simulink library "ammclib_bam_S32K3xx"  (R2016a)
(part 17 of 50)

      |   f32RampUp=round(rampsc*2^31);
      |   if f32RampUp>2^31-1
      |     f32RampUp=2^31-1;
      |     warning(['Parameter f32RampUp of ' gcb ' exceeds the fixed-point range.']);
      |   end
      |   if f32RampUp<-2^31
      |     f32RampUp=-2^31;
      |     warning(['Parameter f32RampUp of ' gcb ' exceeds the fixed-point range.']);
      |   end
      |   f32RampDown=round(rampsc*2^31);
      |   if f32RampDown>2^31-1
      |     f32RampDown=2^31-1;
      |     warning(['Parameter f32RampDown of ' gcb ' exceeds the fixed-point range.']);
      |   end
      |   if f32RampDown<-2^31
      |     f32RampDown=-2^31;
      |     warning(['Parameter f32RampDown of ' gcb ' exceeds the fixed-point range.']);
      |   end
      |   if isnan(u16NSamplesW)
      |     if ~strcmp(u16NSamplesW_bkup,'0')
      |       set_param(gcb,'u16NSamplesW','0');
      |     end
      |   else
      |     tmps=num2str(u16NSamplesW);
      |     if ~strcmp(u16NSamplesW_bkup,tmps)
      |       set_param(gcb,'u16NSamplesW',tmps);
      |     end
      |   end
      |   if isnan(u16NSamplesFW)
      |     if ~strcmp(u16NSamplesFW_bkup,'0')
      |       set_param(gcb,'u16NSamplesFW','0');
      |     end
      |   else
      |     tmps=num2str(u16NSamplesFW);
      |     if ~strcmp(u16NSamplesFW_bkup,tmps)
      |       set_param(gcb,'u16NSamplesFW',tmps);
      |     end
      |   end
      |   if isnan(f32PropGainQ)
      |     if ~strcmp(f32PropGainQ_bkup,'0')
      |       set_param(gcb,'f32PropGainQ','0');
      |     end
      |   else
      |     tmps=num2str(f32PropGainQ);
      |     if ~strcmp(f32PropGainQ_bkup,tmps)
      |       set_param(gcb,'f32PropGainQ',tmps);
      |     end
      |   end
      |   if isnan(f32IntegGainQ)
      |     if ~strcmp(f32IntegGainQ_bkup,'0')
      |       set_param(gcb,'f32IntegGainQ','0');
      |     end
      |   else
      |     tmps=num2str(f32IntegGainQ);
      |     if ~strcmp(f32IntegGainQ_bkup,tmps)
      |       set_param(gcb,'f32IntegGainQ',tmps);
      |     end
      |   end
      |   if isnan(s16PropGainShiftQ)
      |     if ~strcmp(s16PropGainShiftQ_bkup,'0')
      |       set_param(gcb,'s16PropGainShiftQ','0');
      |     end
      |   else
      |     tmps=num2str(s16PropGainShiftQ);
      |     if ~strcmp(s16PropGainShiftQ_bkup,tmps)
      |       set_param(gcb,'s16PropGainShiftQ',tmps);
      |     end
      |   end
      |   if isnan(s16IntegGainShiftQ)
      |     if ~strcmp(s16IntegGainShiftQ_bkup,'0')
      |       set_param(gcb,'s16IntegGainShiftQ','0');
      |     end
      |   else
      |     tmps=num2str(s16IntegGainShiftQ);
      |     if ~strcmp(s16IntegGainShiftQ_bkup,tmps)
      |       set_param(gcb,'s16IntegGainShiftQ',tmps);
      |     end
      |   end
      |   if isnan(f32LowerLimitQ)
      |     if ~strcmp(f32LowerLimitQ_bkup,'0')
      |       set_param(gcb,'f32LowerLimitQ','0');
      |     end
      |   else
      |     tmps=num2str(f32LowerLimitQ);
      |     if ~strcmp(f32LowerLimitQ_bkup,tmps)
      |       set_param(gcb,'f32LowerLimitQ',tmps);
      |     end
      |   end
      |   if isnan(f32UpperLimitQ)
      |     if ~strcmp(f32UpperLimitQ_bkup,'0')
      |       set_param(gcb,'f32UpperLimitQ','0');
      |     end
      |   else
      |     tmps=num2str(f32UpperLimitQ);
      |     if ~strcmp(f32UpperLimitQ_bkup,tmps)
      |       set_param(gcb,'f32UpperLimitQ',tmps);
      |     end
      |   end
      |   if isnan(f32PropGainFW)
      |     if ~strcmp(f32PropGainFW_bkup,'0')
      |       set_param(gcb,'f32PropGainFW','0');
      |     end
      |   else
      |     tmps=num2str(f32PropGainFW);
      |     if ~strcmp(f32PropGainFW_bkup,tmps)
      |       set_param(gcb,'f32PropGainFW',tmps);
      |     end
      |   end
      |   if isnan(f32IntegGainFW)
      |     if ~strcmp(f32IntegGainFW_bkup,'0')
      |       set_param(gcb,'f32IntegGainFW','0');
      |     end
      |   else
      |     tmps=num2str(f32IntegGainFW);
      |     if ~strcmp(f32IntegGainFW_bkup,tmps)
      |       set_param(gcb,'f32IntegGainFW',tmps);
      |     end
      |   end
      |   if isnan(s16PropGainShiftFW)
      |     if ~strcmp(s16PropGainShiftFW_bkup,'0')
      |       set_param(gcb,'s16PropGainShiftFW','0');
      |     end
      |   else
      |     tmps=num2str(s16PropGainShiftFW);
      |     if ~strcmp(s16PropGainShiftFW_bkup,tmps)
      |       set_param(gcb,'s16PropGainShiftFW',tmps);
      |     end
      |   end
      |   if isnan(s16IntegGainShiftFW)
      |     if ~strcmp(s16IntegGainShiftFW_bkup,'0')
      |       set_param(gcb,'s16IntegGainShiftFW','0');
      |     end
      |   else
      |     tmps=num2str(s16IntegGainShiftFW);
      |     if ~strcmp(s16IntegGainShiftFW_bkup,tmps)
      |       set_param(gcb,'s16IntegGainShiftFW',tmps);
      |     end
      |   end
      |   if isnan(f32LowerLimitFW)
      |     if ~strcmp(f32LowerLimitFW_bkup,'0')
      |       set_param(gcb,'f32LowerLimitFW','0');
      |     end
      |   else
      |     tmps=num2str(f32LowerLimitFW);
      |     if ~strcmp(f32LowerLimitFW_bkup,tmps)
      |       set_param(gcb,'f32LowerLimitFW',tmps);
      |     end
      |   end
      |   if isnan(f32UpperLimitFW)
      |     if ~strcmp(f32UpperLimitFW_bkup,'0')
      |       set_param(gcb,'f32UpperLimitFW','0');
      |     end
      |   else
      |     tmps=num2str(f32UpperLimitFW);
      |     if ~strcmp(f32UpperLimitFW_bkup,tmps)
      |       set_param(gcb,'f32UpperLimitFW',tmps);
      |     end
      |   end
      |   if isnan(f32RampUp)
      |     if ~strcmp(f32RampUp_bkup,'0')
      |       set_param(gcb,'f32RampUp','0');
      |     end
      |   else
      |     tmps=num2str(f32RampUp);
      |     if ~strcmp(f32RampUp_bkup,tmps)
      |       set_param(gcb,'f32RampUp',tmps);
      |     end
      |   end
      |   if isnan(f32RampDown)
      |     if ~strcmp(f32RampDown_bkup,'0')
      |       set_param(gcb,'f32RampDown','0');
      |     end
      |   else
      |     tmps=num2str(f32RampDown);
      |     if ~strcmp(f32RampDown_bkup,tmps)
      |       set_param(gcb,'f32RampDown',tmps);
      |     end
      |   end
      | end
      mask Callback autoCalcEn:
      | maskStr=get_param(gcb,'showStates');
      | if strcmp(maskStr,'Hide (faster execution)')
      |   p=Simulink.Mask.get(gcb);
      |   autoCalcEn=get_param(gcb,'autoCalcEn');
      |   hintText=p.getDialogControl('timeHint');
      |   if strcmp(autoCalcEn,'on')
      |     param=p.getParameter('iscale');
      |     if strcmp(param.Enabled,'off')
      |       SampleTime=Simulink.data.evalinGlobal(bdroot,get_param(gcb,'SampleTime'));
      |       if SampleTime==-1
      |         SampleTime=str2double(get_param(gcb,'SampleTime_1'));
      |         if isnan(SampleTime)
      |           hintText.Prompt=['Note: Implementation parameters cannot be calculated yet because the block''s inherited sample time is unknown. Simulink will update the sample time when you run the simulation.'];
      |         else
      |           hintText.Prompt=['Caution: Implementation parameters depend on inherited sample time. Make sure that the sample time of the block''s inputs corresponds to the sampling period in the target application.'];
      |         end
      |       else
      |         hintText.Prompt='Caution: Implementation parameters depend on the sample time. Make sure that the simulation time step corresponds to the sampling period in the target application.';
      |       end
      |       p=Simulink.Mask.get(gcb);
      |       param=p.getParameter('wf0');
      |       param.set('Enabled','on');
      |       param=p.getParameter('wksi');
      |       param.set('Enabled','on');
      |       param=p.getParameter('J');
      |       param.set('Enabled','on');
      |       param=p.getParameter('Kt');
      |       param.set('Enabled','on');
      |       param=p.getParameter('lambdaW');
      |       param.set('Enabled','on');
      |       param=p.getParameter('lambdaFW');
      |       param.set('Enabled','on');
      |       param=p.getParameter('Idmax');
      |       param.set('Enabled','on');
      |       param=p.getParameter('ramprpm');
      |       param.set('Enabled','on');
      |       param=p.getParameter('mechspeed');
      |       param.set('Enabled','on');
      |       param=p.getParameter('polepairs');
      |       param.set('Enabled','on');
      |       param=p.getParameter('uscale');
      |       param.set('Enabled','on');
      |       param=p.getParameter('iscale');
      |       param.set('Enabled','on');
      |     else
      |       SampleTime=Simulink.data.evalinGlobal(bdroot,get_param(gcb,'SampleTime'));
      |       if SampleTime==-1
      |         SampleTime=str2double(get_param(gcb,'SampleTime_1'));
      |       end
      |     end
      |     u16NSamplesW_bkup=get_param(gcb,'u16NSamplesW');
      |     u16NSamplesFW_bkup=get_param(gcb,'u16NSamplesFW');
      |     f32PropGainQ_bkup=get_param(gcb,'f32PropGainQ');
      |     f32IntegGainQ_bkup=get_param(gcb,'f32IntegGainQ');
      |     s16PropGainShiftQ_bkup=get_param(gcb,'s16PropGainShiftQ');
      |     s16IntegGainShiftQ_bkup=get_param(gcb,'s16IntegGainShiftQ');
      |     f32LowerLimitQ_bkup=get_param(gcb,'f32LowerLimitQ');
      |     f32UpperLimitQ_bkup=get_param(gcb,'f32UpperLimitQ');
      |     f32PropGainFW_bkup=get_param(gcb,'f32PropGainFW');
      |     f32IntegGainFW_bkup=get_param(gcb,'f32IntegGainFW');
      |     s16PropGainShiftFW_bkup=get_param(gcb,'s16PropGainShiftFW');
      |     s16IntegGainShiftFW_bkup=get_param(gcb,'s16IntegGainShiftFW');
      |     f32LowerLimitFW_bkup=get_param(gcb,'f32LowerLimitFW');
      |     f32UpperLimitFW_bkup=get_param(gcb,'f32UpperLimitFW');
      |     f32RampUp_bkup=get_param(gcb,'f32RampUp');
      |     f32RampDown_bkup=get_param(gcb,'f32RampDown');
      |     wf0=Simulink.data.evalinGlobal(bdroot,get_param(gcb,'wf0'));
      |     wksi=Simulink.data.evalinGlobal(bdroot,get_param(gcb,'wksi'));
      |     J=Simulink.data.evalinGlobal(bdroot,get_param(gcb,'J'));
      |     Kt=Simulink.data.evalinGlobal(bdroot,get_param(gcb,'Kt'));
      |     lambdaW=Simulink.data.evalinGlobal(bdroot,get_param(gcb,'lambdaW'));
      |     lambdaFW=Simulink.data.evalinGlobal(bdroot,get_param(gcb,'lambdaFW'));
      |     Idmax=Simulink.data.evalinGlobal(bdroot,get_param(gcb,'Idmax'));
      |     ramprpm=Simulink.data.evalinGlobal(bdroot,get_param(gcb,'ramprpm'));
      |     mechspeed=Simulink.data.evalinGlobal(bdroot,get_param(gcb,'mechspeed'));
      |     polepairs=Simulink.data.evalinGlobal(bdroot,get_param(gcb,'polepairs'));
      |     uscale=Simulink.data.evalinGlobal(bdroot,get_param(gcb,'uscale'));
      |     iscale=Simulink.data.evalinGlobal(bdroot,get_param(gcb,'iscale'));
      |     if (wf0<=0)
      |       warning('Natural frequency f0 must be positive.');
      |     end
      |     if (wksi<=0)
      |       warning('Current loop attenuation must be positive.');
      |     end
      |     if (wksi>1)
      |       warning('Current loop attenuation must not exceed 1.');
      |     end
      |     if (J<=0)
      |       warning('Moment of inertia J must be positive.');
      |     end
      |     if (Kt<=0)
      |       warning('Torque constant Kt must be positive.');
      |     end
      |     if (lambdaW<0)
      |       warning('MA filter smoothing factor must be in the range 0..1.');
      |     end
      |     if (lambdaW>1)
      |       warning('MA filter smoothing factor must be in the range 0..1.');
      |     end
      |     if (lambdaFW<0)
      |       warning('MA filter smoothing factor must be in the range 0..1.');
      |     end
      |     if (lambdaFW>1)
      |       warning('MA filter smoothing factor must be in the range 0..1.');
      |     end
      |     if (mechspeed<=0)
      |       warning('Max. speed must be positive.');
      |     end
      |     if (polepairs<1)
      |       warning('Number of pole pairs must be a natural number (1, 2, 3, ...).');
      |     end
      |     if (round(polepairs)~=polepairs)
      |       warning('Number of pole pairs must be a natural number (1, 2, 3, ...).');
      |     end
      |     if (uscale<=0)
      |       warning('U_max must be positive.');
      |     end
      |     if (iscale<=0)
      |       warning('I_max must be positive.');
      |     end
      |     w0=6.283185307179586*wf0;
      |     pgain=2.0*wksi*w0*J/Kt;
      |     igain=w0*w0*J/Kt;
      |     wmax=polepairs*mechspeed*0.1047197551196598;
      |     kpf=pgain*wmax/iscale;
      |     s16PropGainShiftQ=ceil(log2(abs(kpf)));
      |     if s16PropGainShiftQ<-31
      |       s16PropGainShiftQ=-31;
      |     end
      |     if s16PropGainShiftQ>31
      |       s16PropGainShiftQ=31;
      |       warning(['Parameter s16PropGainShiftQ of ' gcb ' exceeds the fixed-point range.']);
      |     end
      |     f32PropGainQ=round(kpf*2^(-s16PropGainShiftQ)*2^31);
      |     if f32PropGainQ>2^31-1
      |       f32PropGainQ=2^31-1;
      |       warning(['Parameter f32PropGainQ of ' gcb ' exceeds the fixed-point range.']);
      |     end
      |     if f32PropGainQ<-2^31
      |       f32PropGainQ=-2^31;
      |       warning(['Parameter f32PropGainQ of ' gcb ' exceeds the fixed-point range.']);
      |     end
      |     kif=igain*SampleTime*0.5*wmax/iscale;
      |     s16IntegGainShiftQ=ceil(log2(abs(kif)));
      |     if s16IntegGainShiftQ<-31
      |       s16IntegGainShiftQ=-31;
      |     end
      |     if s16IntegGainShiftQ>31
      |       s16IntegGainShiftQ=31;
      |       warning(['Parameter s16IntegGainShiftQ of ' gcb ' exceeds the fixed-point range.']);
      |     end
      |     f32IntegGainQ=round(kif*2^(-s16IntegGainShiftQ)*2^31);
      |     if f32IntegGainQ>2^31-1
      |       f32IntegGainQ=2^31-1;
      |       warning(['Parameter f32IntegGainQ of ' gcb ' exceeds the fixed-point range.']);
      |     end
      |     if f32IntegGainQ<-2^31
      |       f32IntegGainQ=-2^31;
      |       warning(['Parameter f32IntegGainQ of ' gcb ' exceeds the fixed-point range.']);
      |     end
      |     f32LowerLimitQ=-2147483648;
      |     f32UpperLimitQ=2147483647;
      |     fwkpf=0.9*pgain*wmax/iscale;
      |     s16PropGainShiftFW=ceil(log2(abs(fwkpf)));
      |     if s16PropGainShiftFW<-31
      |       s16PropGainShiftFW=-31;
      |     end
      |     if s16PropGainShiftFW>31
      |       s16PropGainShiftFW=31;
      |       warning(['Parameter s16PropGainShiftFW of ' gcb ' exceeds the fixed-point range.']);
      |     end
      |     f32PropGainFW=round(fwkpf*2^(-s16PropGainShiftFW)*2^31);
      |     if f32PropGainFW>2^31-1
      |       f32PropGainFW=2^31-1;
      |       warning(['Parameter f32PropGainFW of ' gcb ' exceeds the fixed-point range.']);
      |     end
      |     if f32PropGainFW<-2^31
      |       f32PropGainFW=-2^31;
      |       warning(['Parameter f32PropGainFW of ' gcb ' exceeds the fixed-point range.']);
      |     end
      |     s16IntegGainShiftFW=s16IntegGainShiftQ;
      |     f32IntegGainFW=f32IntegGainQ;
      |     if (Idmax<0)
      |       iratio=abs(Idmax)/iscale;
      |       if (abs(iratio) > 1)
      |         iratio = 0;
      |       end
      |       lowlim=0.3183098861837907*acos(iratio)-0.5;
      |     else
      |       lowlim=0.0;
      |     end
      |     f32LowerLimitFW=round(lowlim*2^31);
      |     if f32LowerLimitFW>2^31-1
      |       f32LowerLimitFW=2^31-1;
      |       warning(['Parameter f32LowerLimitFW of ' gcb ' exceeds the fixed-point range.']);
      |     end
      |     if f32LowerLimitFW<-2^31
      |       f32LowerLimitFW=-2^31;
      |       warning(['Parameter f32LowerLimitFW of ' gcb ' exceeds the fixed-point range.']);
      |     end
      |     f32UpperLimitFW=0;
      |     u16NSamplesW=round(log2(1.0/abs(lambdaW)));
      |     if u16NSamplesW>31
      |       u16NSamplesW=31;
      |     end
      |     if u16NSamplesW<0
      |       u16NSamplesW=0;
      |     end
      |     u16NSamplesFW=round(log2(1.0/abs(lambdaFW)));
      |     if u16NSamplesFW>31
      |       u16NSamplesFW=31;
      |     end
      |     if u16NSamplesFW<0
      |       u16NSamplesFW=0;
      |     end
      |     rampsc=polepairs*abs(ramprpm)*0.1047197551196598/wmax;
      |     f32RampUp=round(rampsc*2^31);
      |     if f32RampUp>2^31-1
      |       f32RampUp=2^31-1;
      |       warning(['Parameter f32RampUp of ' gcb ' exceeds the fixed-point range.']);
      |     end
      |     if f32RampUp<-2^31
      |       f32RampUp=-2^31;
      |       warning(['Parameter f32RampUp of ' gcb ' exceeds the fixed-point range.']);
      |     end
      |     f32RampDown=round(rampsc*2^31);
      |     if f32RampDown>2^31-1
      |       f32RampDown=2^31-1;
      |       warning(['Parameter f32RampDown of ' gcb ' exceeds the fixed-point range.']);
      |     end
      |     if f32RampDown<-2^31
      |       f32RampDown=-2^31;
      |       warning(['Parameter f32RampDown of ' gcb ' exceeds the fixed-point range.']);
      |     end
      |     if isnan(u16NSamplesW)
      |       if ~strcmp(u16NSamplesW_bkup,'0')
      |         set_param(gcb,'u16NSamplesW','0');
      |       end
      |     else
      |       tmps=num2str(u16NSamplesW);
      |       if ~strcmp(u16NSamplesW_bkup,tmps)
      |         set_param(gcb,'u16NSamplesW',tmps);
      |       end
      |     end
      |     if isnan(u16NSamplesFW)
      |       if ~strcmp(u16NSamplesFW_bkup,'0')
      |         set_param(gcb,'u16NSamplesFW','0');
      |       end
      |     else
      |       tmps=num2str(u16NSamplesFW);
      |       if ~strcmp(u16NSamplesFW_bkup,tmps)
      |         set_param(gcb,'u16NSamplesFW',tmps);
      |       end
      |     end
      |     if isnan(f32PropGainQ)
      |       if ~strcmp(f32PropGainQ_bkup,'0')
      |         set_param(gcb,'f32PropGainQ','0');
      |       end
      |     else
      |       tmps=num2str(f32PropGainQ);
      |       if ~strcmp(f32PropGainQ_bkup,tmps)
      |         set_param(gcb,'f32PropGainQ',tmps);
      |       end
      |     end
      |     if isnan(f32IntegGainQ)
      |       if ~strcmp(f32IntegGainQ_bkup,'0')
      |         set_param(gcb,'f32IntegGainQ','0');
      |       end
      |     else
      |       tmps=num2str(f32IntegGainQ);
      |       if ~strcmp(f32IntegGainQ_bkup,tmps)
      |         set_param(gcb,'f32IntegGainQ',tmps);
      |       end
      |     end
      |     if isnan(s16PropGainShiftQ)
      |       if ~strcmp(s16PropGainShiftQ_bkup,'0')
      |         set_param(gcb,'s16PropGainShiftQ','0');
      |       end
      |     else
      |       tmps=num2str(s16PropGainShiftQ);
      |       if ~strcmp(s16PropGainShiftQ_bkup,tmps)
      |         set_param(gcb,'s16PropGainShiftQ',tmps);
      |       end
      |     end
      |     if isnan(s16IntegGainShiftQ)
      |       if ~strcmp(s16IntegGainShiftQ_bkup,'0')
      |         set_param(gcb,'s16IntegGainShiftQ','0');
      |       end
      |     else
      |       tmps=num2str(s16IntegGainShiftQ);
      |       if ~strcmp(s16IntegGainShiftQ_bkup,tmps)
      |         set_param(gcb,'s16IntegGainShiftQ',tmps);
      |       end
      |     end
      |     if isnan(f32LowerLimitQ)
      |       if ~strcmp(f32LowerLimitQ_bkup,'0')
      |         set_param(gcb,'f32LowerLimitQ','0');
      |       end
      |     else
      |       tmps=num2str(f32LowerLimitQ);
      |       if ~strcmp(f32LowerLimitQ_bkup,tmps)
      |         set_param(gcb,'f32LowerLimitQ',tmps);
      |       end
      |     end
      |     if isnan(f32UpperLimitQ)
      |       if ~strcmp(f32UpperLimitQ_bkup,'0')
      |         set_param(gcb,'f32UpperLimitQ','0');
      |       end
      |     else
      |       tmps=num2str(f32UpperLimitQ);
      |       if ~strcmp(f32UpperLimitQ_bkup,tmps)
      |         set_param(gcb,'f32UpperLimitQ',tmps);
      |       end
      |     end
      |     if isnan(f32PropGainFW)
      |       if ~strcmp(f32PropGainFW_bkup,'0')
      |         set_param(gcb,'f32PropGainFW','0');
      |       end
      |     else
      |       tmps=num2str(f32PropGainFW);
      |       if ~strcmp(f32PropGainFW_bkup,tmps)
      |         set_param(gcb,'f32PropGainFW',tmps);
      |       end
      |     end
      |     if isnan(f32IntegGainFW)
      |       if ~strcmp(f32IntegGainFW_bkup,'0')
      |         set_param(gcb,'f32IntegGainFW','0');
      |       end
      |     else
      |       tmps=num2str(f32IntegGainFW);
      |       if ~strcmp(f32IntegGainFW_bkup,tmps)
      |         set_param(gcb,'f32IntegGainFW',tmps);
      |       end
      |     end
      |     if isnan(s16PropGainShiftFW)
      |       if ~strcmp(s16PropGainShiftFW_bkup,'0')
      |         set_param(gcb,'s16PropGainShiftFW','0');
      |       end
      |     else
      |       tmps=num2str(s16PropGainShiftFW);
      |       if ~strcmp(s16PropGainShiftFW_bkup,tmps)
      |         set_param(gcb,'s16PropGainShiftFW',tmps);
      |       end
      |     end
      |     if isnan(s16IntegGainShiftFW)
      |       if ~strcmp(s16IntegGainShiftFW_bkup,'0')
      |         set_param(gcb,'s16IntegGainShiftFW','0');
      |       end
      |     else
      |       tmps=num2str(s16IntegGainShiftFW);
      |       if ~strcmp(s16IntegGainShiftFW_bkup,tmps)
      |         set_param(gcb,'s16IntegGainShiftFW',tmps);
      |       end
      |     end
      |     if isnan(f32LowerLimitFW)
      |       if ~strcmp(f32LowerLimitFW_bkup,'0')
      |         set_param(gcb,'f32LowerLimitFW','0');
      |       end
      |     else
      |       tmps=num2str(f32LowerLimitFW);
      |       if ~strcmp(f32LowerLimitFW_bkup,tmps)
      |         set_param(gcb,'f32LowerLimitFW',tmps);
      |       end
      |     end
      |     if isnan(f32UpperLimitFW)
      |       if ~strcmp(f32UpperLimitFW_bkup,'0')
      |         set_param(gcb,'f32UpperLimitFW','0');
      |       end
      |     else
      |       tmps=num2str(f32UpperLimitFW);
      |       if ~strcmp(f32UpperLimitFW_bkup,tmps)
      |         set_param(gcb,'f32UpperLimitFW',tmps);
      |       end
      |     end
      |     if isnan(f32RampUp)
      |       if ~strcmp(f32RampUp_bkup,'0')
      |         set_param(gcb,'f32RampUp','0');
      |       end
      |     else
      |       tmps=num2str(f32RampUp);
      |       if ~strcmp(f32RampUp_bkup,tmps)
      |         set_param(gcb,'f32RampUp',tmps);
      |       end
      |     end
      |     if isnan(f32RampDown)
      |       if ~strcmp(f32RampDown_bkup,'0')
      |         set_param(gcb,'f32RampDown','0');
      |       end
      |     else
      |       tmps=num2str(f32RampDown);
      |       if ~strcmp(f32RampDown_bkup,tmps)
      |         set_param(gcb,'f32RampDown',tmps);
      |       end
      |     end
      |   else
      |     param=p.getParameter('iscale');
      |     if strcmp(param.Enabled,'on')
      |       hintText.Prompt='Caution: Implementation parameters are fixed.';
      |       p=Simulink.Mask.get(gcb);
      |       param=p.getParameter('wf0');
      |       param.set('Enabled','off');
      |       param=p.getParameter('wksi');
      |       param.set('Enabled','off');
      |       param=p.getParameter('J');
      |       param.set('Enabled','off');
      |       param=p.getParameter('Kt');
      |       param.set('Enabled','off');
      |       param=p.getParameter('lambdaW');
      |       param.set('Enabled','off');
      |       param=p.getParameter('lambdaFW');
      |       param.set('Enabled','off');
      |       param=p.getParameter('Idmax');
      |       param.set('Enabled','off');
      |       param=p.getParameter('ramprpm');
      |       param.set('Enabled','off');
      |       param=p.getParameter('mechspeed');
      |       param.set('Enabled','off');
      |       param=p.getParameter('polepairs');
      |       param.set('Enabled','off');
      |       param=p.getParameter('uscale');
      |       param.set('Enabled','off');
      |       param=p.getParameter('iscale');
      |       param.set('Enabled','off');
      |     end
      |   end
      | end
      mask DialogControl CompBut Prompt: Recalculate sample times
      mask DialogControl CompBut Tooltip: Simulink updates the sample times of all blocks when the simulation is run. This button will update the sample times now.
      mask DialogControl CompBut Callback:
      | btn=questdlg('This will apply all changes in all open dialog boxes and update the schematic. Do you want to proceed?','Apply all changes','Continue','Cancel','Continue');
      | if strcmp(btn,'Continue')
      |   dlgs=DAStudio.ToolRoot.getOpenDialogs;
      |   for i=1:length(dlgs)
      |     dlgs(i).apply;
      |   end
      |   try
      |     SampleTime_1=str2double(get_param(gcb,'SampleTime_1'));
      |     ts=Simulink.Block.getSampleTimes(gcb);
      |     ts=ts(1).Value(1);
      |     if (SampleTime_1 ~= ts)
      |       SampleTime_1=ts;
      |       set_param(gcb,'SampleTime_1',num2str(ts));
      |       autoCalcEn=get_param(gcb,'autoCalcEn');
      |       if strcmp(autoCalcEn,'on')
      |         SampleTime=Simulink.data.evalinGlobal(bdroot,get_param(gcb,'SampleTime'));
      |         p=Simulink.Mask.get(gcb);
      |         hintText=p.getDialogControl('timeHint');
      |         if SampleTime==-1
      |           SampleTime=SampleTime_1;
      |           hintText.Prompt='Caution: Implementation parameters depend on inherited sample time. Make sure that the sample time of the block''s inputs corresponds to the sampling period in the target application.';
      |         else
      |           hintText.Prompt='Caution: Implementation parameters depend on the sample time. Make sure that the simulation time step corresponds to the sampling period in the target application.';
      |         end
      |         u16NSamplesW_bkup=get_param(gcb,'u16NSamplesW');
      |         u16NSamplesFW_bkup=get_param(gcb,'u16NSamplesFW');
      |         f32PropGainQ_bkup=get_param(gcb,'f32PropGainQ');
      |         f32IntegGainQ_bkup=get_param(gcb,'f32IntegGainQ');
      |         s16PropGainShiftQ_bkup=get_param(gcb,'s16PropGainShiftQ');
      |         s16IntegGainShiftQ_bkup=get_param(gcb,'s16IntegGainShiftQ');
      |         f32LowerLimitQ_bkup=get_param(gcb,'f32LowerLimitQ');
      |         f32UpperLimitQ_bkup=get_param(gcb,'f32UpperLimitQ');
      |         f32PropGainFW_bkup=get_param(gcb,'f32PropGainFW');
      |         f32IntegGainFW_bkup=get_param(gcb,'f32IntegGainFW');
      |         s16PropGainShiftFW_bkup=get_param(gcb,'s16PropGainShiftFW');
      |         s16IntegGainShiftFW_bkup=get_param(gcb,'s16IntegGainShiftFW');
      |         f32LowerLimitFW_bkup=get_param(gcb,'f32LowerLimitFW');
      |         f32UpperLimitFW_bkup=get_param(gcb,'f32UpperLimitFW');
      |         f32RampUp_bkup=get_param(gcb,'f32RampUp');
      |         f32RampDown_bkup=get_param(gcb,'f32RampDown');
      |         wf0=Simulink.data.evalinGlobal(bdroot,get_param(gcb,'wf0'));
      |         wksi=Simulink.data.evalinGlobal(bdroot,get_param(gcb,'wksi'));
      |         J=Simulink.data.evalinGlobal(bdroot,get_param(gcb,'J'));
      |         Kt=Simulink.data.evalinGlobal(bdroot,get_param(gcb,'Kt'));
      |         lambdaW=Simulink.data.evalinGlobal(bdroot,get_param(gcb,'lambdaW'));
      |         lambdaFW=Simulink.data.evalinGlobal(bdroot,get_param(gcb,'lambdaFW'));
      |         Idmax=Simulink.data.evalinGlobal(bdroot,get_param(gcb,'Idmax'));
      |         ramprpm=Simulink.data.evalinGlobal(bdroot,get_param(gcb,'ramprpm'));
      |         mechspeed=Simulink.data.evalinGlobal(bdroot,get_param(gcb,'mechspeed'));
      |         polepairs=Simulink.data.evalinGlobal(bdroot,get_param(gcb,'polepairs'));
      |         uscale=Simulink.data.evalinGlobal(bdroot,get_param(gcb,'uscale'));
      |         iscale=Simulink.data.evalinGlobal(bdroot,get_param(gcb,'iscale'));
      |         if (wf0<=0)
      |           warning('Natural frequency f0 must be positive.');
      |         end
      |         if (wksi<=0)
      |           warning('Current loop attenuation must be positive.');
      |         end
      |         if (wksi>1)
      |           warning('Current loop attenuation must not exceed 1.');
      |         end
      |         if (J<=0)
      |           warning('Moment of inertia J must be positive.');
      |         end
      |         if (Kt<=0)
      |           warning('Torque constant Kt must be positive.');
      |         end
      |         if (lambdaW<0)
      |           warning('MA filter smoothing factor must be in the range 0..1.');
      |         end
      |         if (lambdaW>1)
      |           warning('MA filter smoothing factor must be in the range 0..1.');
      |         end
      |         if (lambdaFW<0)
      |           warning('MA filter smoothing factor must be in the range 0..1.');
      |         end
      |         if (lambdaFW>1)
      |           warning('MA filter smoothing factor must be in the range 0..1.');
      |         end
      |         if (mechspeed<=0)
      |           warning('Max. speed must be positive.');
      |         end
      |         if (polepairs<1)
      |           warning('Number of pole pairs must be a natural number (1, 2, 3, ...).');
      |         end
      |         if (round(polepairs)~=polepairs)
      |           warning('Number of pole pairs must be a natural number (1, 2, 3, ...).');
      |         end
      |         if (uscale<=0)
      |           warning('U_max must be positive.');
      |         end
      |         if (iscale<=0)
      |           warning('I_max must be positive.');
      |         end
      |         w0=6.283185307179586*wf0;
      |         pgain=2.0*wksi*w0*J/Kt;
      |         igain=w0*w0*J/Kt;
      |         wmax=polepairs*mechspeed*0.1047197551196598;
      |         kpf=pgain*wmax/iscale;
      |         s16PropGainShiftQ=ceil(log2(abs(kpf)));
      |         if s16PropGainShiftQ<-31
      |           s16PropGainShiftQ=-31;
      |         end
      |         if s16PropGainShiftQ>31
      |           s16PropGainShiftQ=31;
      |           warning(['Parameter s16PropGainShiftQ of ' gcb ' exceeds the fixed-point range.']);
      |         end
      |         f32PropGainQ=round(kpf*2^(-s16PropGainShiftQ)*2^31);
      |         if f32PropGainQ>2^31-1
      |           f32PropGainQ=2^31-1;
      |           warning(['Parameter f32PropGainQ of ' gcb ' exceeds the fixed-point range.']);
      |         end
      |         if f32PropGainQ<-2^31
      |           f32PropGainQ=-2^31;
      |           warning(['Parameter f32PropGainQ of ' gcb ' exceeds the fixed-point range.']);
      |         end
      |         kif=igain*SampleTime*0.5*wmax/iscale;
      |         s16IntegGainShiftQ=ceil(log2(abs(kif)));
      |         if s16IntegGainShiftQ<-31
      |           s16IntegGainShiftQ=-31;
      |         end
      |         if s16IntegGainShiftQ>31
      |           s16IntegGainShiftQ=31;
      |           warning(['Parameter s16IntegGainShiftQ of ' gcb ' exceeds the fixed-point range.']);
      |         end
      |         f32IntegGainQ=round(kif*2^(-s16IntegGainShiftQ)*2^31);
      |         if f32IntegGainQ>2^31-1
      |           f32IntegGainQ=2^31-1;
      |           warning(['Parameter f32IntegGainQ of ' gcb ' exceeds the fixed-point range.']);
      |         end
      |         if f32IntegGainQ<-2^31
      |           f32IntegGainQ=-2^31;
      |           warning(['Parameter f32IntegGainQ of ' gcb ' exceeds the fixed-point range.']);
      |         end
      |         f32LowerLimitQ=-2147483648;
      |         f32UpperLimitQ=2147483647;
      |         fwkpf=0.9*pgain*wmax/iscale;
      |         s16PropGainShiftFW=ceil(log2(abs(fwkpf)));
      |         if s16PropGainShiftFW<-31
      |           s16PropGainShiftFW=-31;
      |         end
      |         if s16PropGainShiftFW>31
      |           s16PropGainShiftFW=31;
      |           warning(['Parameter s16PropGainShiftFW of ' gcb ' exceeds the fixed-point range.']);
      |         end
      |         f32PropGainFW=round(fwkpf*2^(-s16PropGainShiftFW)*2^31);
      |         if f32PropGainFW>2^31-1
      |           f32PropGainFW=2^31-1;
      |           warning(['Parameter f32PropGainFW of ' gcb ' exceeds the fixed-point range.']);
      |         end
      |         if f32PropGainFW<-2^31
      |           f32PropGainFW=-2^31;
      |           warning(['Parameter f32PropGainFW of ' gcb ' exceeds the fixed-point range.']);
      |         end
      |         s16IntegGainShiftFW=s16IntegGainShiftQ;
      |         f32IntegGainFW=f32IntegGainQ;
      |         if (Idmax<0)
      |           iratio=abs(Idmax)/iscale;
      |           if (abs(iratio) > 1)
      |             iratio = 0;
      |           end
      |           lowlim=0.3183098861837907*acos(iratio)-0.5;
      |         else
      |           lowlim=0.0;
      |         end
      |         f32LowerLimitFW=round(lowlim*2^31);
      |         if f32LowerLimitFW>2^31-1
      |           f32LowerLimitFW=2^31-1;
      |           warning(['Parameter f32LowerLimitFW of ' gcb ' exceeds the fixed-point range.']);
      |         end
      |         if f32LowerLimitFW<-2^31
      |           f32LowerLimitFW=-2^31;
      |           warning(['Parameter f32LowerLimitFW of ' gcb ' exceeds the fixed-point range.']);
      |         end
      |         f32UpperLimitFW=0;
      |         u16NSamplesW=round(log2(1.0/abs(lambdaW)));
      |         if u16NSamplesW>31
      |           u16NSamplesW=31;
      |         end
      |         if u16NSamplesW<0
      |           u16NSamplesW=0;
      |         end
      |         u16NSamplesFW=round(log2(1.0/abs(lambdaFW)));
      |         if u16NSamplesFW>31
      |           u16NSamplesFW=31;
      |         end
      |         if u16NSamplesFW<0
      |           u16NSamplesFW=0;
      |         end
      |         rampsc=polepairs*abs(ramprpm)*0.1047197551196598/wmax;
      |         f32RampUp=round(rampsc*2^31);
      |         if f32RampUp>2^31-1
      |           f32RampUp=2^31-1;
      |           warning(['Parameter f32RampUp of ' gcb ' exceeds the fixed-point range.']);
      |         end
      |         if f32RampUp<-2^31
      |           f32RampUp=-2^31;
      |           warning(['Parameter f32RampUp of ' gcb ' exceeds the fixed-point range.']);
      |         end
      |         f32RampDown=round(rampsc*2^31);
      |         if f32RampDown>2^31-1
      |           f32RampDown=2^31-1;
      |           warning(['Parameter f32RampDown of ' gcb ' exceeds the fixed-point range.']);
      |         end
      |         if f32RampDown<-2^31
      |           f32RampDown=-2^31;
      |           warning(['Parameter f32RampDown of ' gcb ' exceeds the fixed-point range.']);
      |         end
      |         if isnan(u16NSamplesW)
      |           if ~strcmp(u16NSamplesW_bkup,'0')
      |             set_param(gcb,'u16NSamplesW','0');
      |           end
      |         else
      |           tmps=num2str(u16NSamplesW);
      |           if ~strcmp(u16NSamplesW_bkup,tmps)
      |             set_param(gcb,'u16NSamplesW',tmps);
      |           end
      |         end
      |         if isnan(u16NSamplesFW)
      |           if ~strcmp(u16NSamplesFW_bkup,'0')
      |             set_param(gcb,'u16NSamplesFW','0');
      |           end
      |         else
      |           tmps=num2str(u16NSamplesFW);
      |           if ~strcmp(u16NSamplesFW_bkup,tmps)
      |             set_param(gcb,'u16NSamplesFW',tmps);
      |           end
      |         end
      |         if isnan(f32PropGainQ)
      |           if ~strcmp(f32PropGainQ_bkup,'0')
      |             set_param(gcb,'f32PropGainQ','0');
      |           end
      |         else
      |           tmps=num2str(f32PropGainQ);
      |           if ~strcmp(f32PropGainQ_bkup,tmps)
      |             set_param(gcb,'f32PropGainQ',tmps);
      |           end
      |         end
      |         if isnan(f32IntegGainQ)
      |           if ~strcmp(f32IntegGainQ_bkup,'0')
      |             set_param(gcb,'f32IntegGainQ','0');
      |           end
      |         else
      |           tmps=num2str(f32IntegGainQ);
      |           if ~strcmp(f32IntegGainQ_bkup,tmps)
      |             set_param(gcb,'f32IntegGainQ',tmps);
      |           end
      |         end
      |         if isnan(s16PropGainShiftQ)
      |           if ~strcmp(s16PropGainShiftQ_bkup,'0')
      |             set_param(gcb,'s16PropGainShiftQ','0');
      |           end
      |         else
      |           tmps=num2str(s16PropGainShiftQ);
      |           if ~strcmp(s16PropGainShiftQ_bkup,tmps)
      |             set_param(gcb,'s16PropGainShiftQ',tmps);
      |           end
      |         end
      |         if isnan(s16IntegGainShiftQ)
      |           if ~strcmp(s16IntegGainShiftQ_bkup,'0')
      |             set_param(gcb,'s16IntegGainShiftQ','0');
      |           end
      |         else
      |           tmps=num2str(s16IntegGainShiftQ);
      |           if ~strcmp(s16IntegGainShiftQ_bkup,tmps)
      |             set_param(gcb,'s16IntegGainShiftQ',tmps);
      |           end
      |         end
      |         if isnan(f32LowerLimitQ)
      |           if ~strcmp(f32LowerLimitQ_bkup,'0')
      |             set_param(gcb,'f32LowerLimitQ','0');
      |           end
      |         else
      |           tmps=num2str(f32LowerLimitQ);
      |           if ~strcmp(f32LowerLimitQ_bkup,tmps)
      |             set_param(gcb,'f32LowerLimitQ',tmps);
      |           end
      |         end
      |         if isnan(f32UpperLimitQ)
      |           if ~strcmp(f32UpperLimitQ_bkup,'0')
      |             set_param(gcb,'f32UpperLimitQ','0');
      |           end
      |         else
      |           tmps=num2str(f32UpperLimitQ);
      |           if ~strcmp(f32UpperLimitQ_bkup,tmps)
      |             set_param(gcb,'f32UpperLimitQ',tmps);
      |           end
      |         end
      |         if isnan(f32PropGainFW)
      |           if ~strcmp(f32PropGainFW_bkup,'0')
      |             set_param(gcb,'f32PropGainFW','0');
      |           end
      |         else
      |           tmps=num2str(f32PropGainFW);
      |           if ~strcmp(f32PropGainFW_bkup,tmps)
      |             set_param(gcb,'f32PropGainFW',tmps);
      |           end
      |         end
      |         if isnan(f32IntegGainFW)
      |           if ~strcmp(f32IntegGainFW_bkup,'0')
      |             set_param(gcb,'f32IntegGainFW','0');
      |           end
      |         else
      |           tmps=num2str(f32IntegGainFW);
      |           if ~strcmp(f32IntegGainFW_bkup,tmps)
      |             set_param(gcb,'f32IntegGainFW',tmps);
      |           end
      |         end
      |         if isnan(s16PropGainShiftFW)
      |           if ~strcmp(s16PropGainShiftFW_bkup,'0')
      |             set_param(gcb,'s16PropGainShiftFW','0');
      |           end
      |         else
      |           tmps=num2str(s16PropGainShiftFW);
      |           if ~strcmp(s16PropGainShiftFW_bkup,tmps)
      |             set_param(gcb,'s16PropGainShiftFW',tmps);
      |           end
      |         end
      |         if isnan(s16IntegGainShiftFW)
      |           if ~strcmp(s16IntegGainShiftFW_bkup,'0')
      |             set_param(gcb,'s16IntegGainShiftFW','0');
      |           end
      |         else
      |           tmps=num2str(s16IntegGainShiftFW);
      |           if ~strcmp(s16IntegGainShiftFW_bkup,tmps)
      |             set_param(gcb,'s16IntegGainShiftFW',tmps);
      |           end
      |         end
      |         if isnan(f32LowerLimitFW)
      |           if ~strcmp(f32LowerLimitFW_bkup,'0')
      |             set_param(gcb,'f32LowerLimitFW','0');
      |           end
      |         else
      |           tmps=num2str(f32LowerLimitFW);
      |           if ~strcmp(f32LowerLimitFW_bkup,tmps)
      |             set_param(gcb,'f32LowerLimitFW',tmps);
      |           end
      |         end
      |         if isnan(f32UpperLimitFW)
      |           if ~strcmp(f32UpperLimitFW_bkup,'0')
      |             set_param(gcb,'f32UpperLimitFW','0');
      |           end
      |         else
      |           tmps=num2str(f32UpperLimitFW);
      |           if ~strcmp(f32UpperLimitFW_bkup,tmps)
      |             set_param(gcb,'f32UpperLimitFW',tmps);
      |           end
      |         end
      |         if isnan(f32RampUp)
      |           if ~strcmp(f32RampUp_bkup,'0')
      |             set_param(gcb,'f32RampUp','0');
      |           end
      |         else
      |           tmps=num2str(f32RampUp);
      |           if ~strcmp(f32RampUp_bkup,tmps)
      |             set_param(gcb,'f32RampUp',tmps);
      |           end
      |         end
      |         if isnan(f32RampDown)
      |           if ~strcmp(f32RampDown_bkup,'0')
      |             set_param(gcb,'f32RampDown','0');
      |           end
      |         else
      |           tmps=num2str(f32RampDown);
      |           if ~strcmp(f32RampDown_bkup,tmps)
      |             set_param(gcb,'f32RampDown',tmps);
      |           end
      |         end
      |       end
      |     end
      |   catch
      |    warning(['Sample time cannot be calculated for the block ' gcb])
      |   end
      | end
      mask DialogControl timeHint Prompt: Note: Implementation parameters cannot be calculated yet because the block's inherited sample time is unknown. Simulink will update the sample time when you run the simulation.
      mask Display:
      | color('black');
      | pos = get_param(gcb, 'Position');
      | width = pos(3) - pos(1);
      | height = pos(4) - pos(2);
      | tX=width/2;
      | tY=height - 25;
      | color('black');
      | text(tX,tY, 'AMCLIB_FWSpeedLoop_F32', 'horizontalAlignment', 'center');
      | if showStates == 2
      |   color('red');
      |   text(tX,tY - 20, ['debugging mode' char(13) char(10) '(limited performance)'], 'horizontalAlignment', 'center');
      | end
  AMCLIB_FW_F32 : Subsystem  StartFcn=|  TreatAsAtomicUnit=on  mask(AMCLIB_FW_F32){showStates=Hide (faster execution), resetStatesEnable=Pre-set according to the first set of inputs after reset, showDebugOutputs=Hide, SampleTime=-1, wf0=30, wksi=1, J=1.6e-5, Kt=0.067, lambdaFW=0.9, Idmax=-5, mechspeed=3000, polepairs=1, uscale=15, iscale=10, autoCalcEn=on, u16NSamples=0, f32PropGain=0, f32IntegGain=0, s16PropGainShift=0, s16IntegGainShift=0, f32LowerLimit=0, f32UpperLimit=0, SampleTime_1=NaN}
      | ts=get_param(gcb,'CompiledSampleTime');
      | if iscell(ts)
      |   ts=ts{1};
      |   if iscell(ts)
      |     ts=ts{1};
      |   end
      | end
      | ts=ts(1);
      | set_param(gcb,'SampleTime_1',num2str(ts));
      | p=Simulink.Mask.get(gcb);
      | hintText=p.getDialogControl('timeHint');
      | SampleTime=Simulink.data.evalinGlobal(bdroot,get_param(gcb,'SampleTime'));
      | p=Simulink.Mask.get(gcb);
      | autoCalcEn=get_param(gcb,'autoCalcEn');
      | if strcmp(autoCalcEn,'on')
      |   if SampleTime==-1
      |     hintText.Prompt='Caution: Implementation parameters depend on inherited sample time. Make sure that the sample time of the block''s inputs corresponds to the sampling period in the target application.';
      |   else
      |     hintText.Prompt='Caution: Implementation parameters depend on the sample time. Make sure that the simulation time step corresponds to the sampling period in the target application.';
      |   end
      |   SampleTime=ts;
      |   u16NSamples_bkup=get_param(gcb,'u16NSamples');
      |   f32PropGain_bkup=get_param(gcb,'f32PropGain');
      |   f32IntegGain_bkup=get_param(gcb,'f32IntegGain');
      |   s16PropGainShift_bkup=get_param(gcb,'s16PropGainShift');
      |   s16IntegGainShift_bkup=get_param(gcb,'s16IntegGainShift');
      |   f32LowerLimit_bkup=get_param(gcb,'f32LowerLimit');
      |   f32UpperLimit_bkup=get_param(gcb,'f32UpperLimit');
      |   wf0=Simulink.data.evalinGlobal(bdroot,get_param(gcb,'wf0'));
      |   wksi=Simulink.data.evalinGlobal(bdroot,get_param(gcb,'wksi'));
      |   J=Simulink.data.evalinGlobal(bdroot,get_param(gcb,'J'));
      |   Kt=Simulink.data.evalinGlobal(bdroot,get_param(gcb,'Kt'));
      |   lambdaFW=Simulink.data.evalinGlobal(bdroot,get_param(gcb,'lambdaFW'));
      |   Idmax=Simulink.data.evalinGlobal(bdroot,get_param(gcb,'Idmax'));
      |   mechspeed=Simulink.data.evalinGlobal(bdroot,get_param(gcb,'mechspeed'));
      |   polepairs=Simulink.data.evalinGlobal(bdroot,get_param(gcb,'polepairs'));
      |   uscale=Simulink.data.evalinGlobal(bdroot,get_param(gcb,'uscale'));
      |   iscale=Simulink.data.evalinGlobal(bdroot,get_param(gcb,'iscale'));
      |   if (wf0<=0)
      |     warning('Natural frequency f0 must be positive.');
      |   end
      |   if (wksi<=0)
      |     warning('Current loop attenuation must be positive.');
      |   end
      |   if (wksi>1)
      |     warning('Current loop attenuation must not exceed 1.');
      |   end
      |   if (J<=0)
      |     warning('Moment of inertia J must be positive.');
      |   end
      |   if (Kt<=0)
      |     warning('Torque constant Kt must be positive.');
      |   end
      |   if (lambdaFW<0)
      |     warning('MA filter smoothing factor must be in the range 0..1.');
      |   end
      |   if (lambdaFW>1)
      |     warning('MA filter smoothing factor must be in the range 0..1.');
      |   end
      |   if (mechspeed<=0)
      |     warning('Max. speed must be positive.');
      |   end
      |   if (polepairs<1)
      |     warning('Number of pole pairs must be a natural number (1, 2, 3, ...).');
      |   end
      |   if (round(polepairs)~=polepairs)
      |     warning('Number of pole pairs must be a natural number (1, 2, 3, ...).');
      |   end
      |   if (uscale<=0)
      |     warning('U_max must be positive.');
      |   end
      |   if (iscale<=0)
      |     warning('I_max must be positive.');
      |   end
      |   w0=6.283185307179586*wf0;
      |   pgain=2.0*wksi*w0*J/Kt;
      |   igain=w0*w0*J/Kt;
      |   wmax=polepairs*mechspeed*0.1047197551196598;
      |   kif=igain*SampleTime*0.5*wmax/iscale;
      |   fwkpf=0.9*pgain*wmax/iscale;
      |   s16PropGainShift=ceil(log2(abs(fwkpf)));
      |   if s16PropGainShift<-31
      |     s16PropGainShift=-31;
      |   end
      |   if s16PropGainShift>31
      |     s16PropGainShift=31;
      |     warning(['Parameter s16PropGainShift of ' gcb ' exceeds the fixed-point range.']);
      |   end
      |   f32PropGain=round(fwkpf*2^(-s16PropGainShift)*2^31);
      |   if f32PropGain>2^31-1
      |     f32PropGain=2^31-1;
      |     warning(['Parameter f32PropGain of ' gcb ' exceeds the fixed-point range.']);
      |   end
      |   if f32PropGain<-2^31
      |     f32PropGain=-2^31;
      |     warning(['Parameter f32PropGain of ' gcb ' exceeds the fixed-point range.']);
      |   end
      |   s16IntegGainShift=ceil(log2(abs(kif)));
      |   if s16IntegGainShift<-31
      |     s16IntegGainShift=-31;
      |   end
      |   if s16IntegGainShift>31
      |     s16IntegGainShift=31;
      |     warning(['Parameter s16IntegGainShift of ' gcb ' exceeds the fixed-point range.']);
      |   end
      |   f32IntegGain=round(kif*2^(-s16IntegGainShift)*2^31);
      |   if f32IntegGain>2^31-1
      |     f32IntegGain=2^31-1;
      |     warning(['Parameter f32IntegGain of ' gcb ' exceeds the fixed-point range.']);
      |   end
      |   if f32IntegGain<-2^31
      |     f32IntegGain=-2^31;
      |     warning(['Parameter f32IntegGain of ' gcb ' exceeds the fixed-point range.']);
      |   end
      |   if (Idmax<0)
      |     iratio=abs(Idmax)/iscale;
      |     lowlim=0.3183098861837907*acos(iratio)-0.5;
      |   else
      |     lowlim=0.0;
      |   end
      |   f32LowerLimit=round(lowlim*2^31);
      |   if f32LowerLimit>2^31-1
      |     f32LowerLimit=2^31-1;
      |     warning(['Parameter f32LowerLimit of ' gcb ' exceeds the fixed-point range.']);
      |   end
      |   if f32LowerLimit<-2^31
      |     f32LowerLimit=-2^31;
      |     warning(['Parameter f32LowerLimit of ' gcb ' exceeds the fixed-point range.']);
      |   end
      |   f32UpperLimit=0;
      |   u16NSamples=round(log2(1.0/abs(lambdaFW)));
      |   if u16NSamples>31
      |     u16NSamples=31;
      |   end
      |   if u16NSamples<0
      |     u16NSamples=0;
      |   end
      |   if isnan(u16NSamples)
      |     if ~strcmp(u16NSamples_bkup,'0')
      |       set_param(gcb,'u16NSamples','0');
      |     end
      |   else
      |     tmps=num2str(u16NSamples);
      |     if ~strcmp(u16NSamples_bkup,tmps)
      |       set_param(gcb,'u16NSamples',tmps);
      |     end
      |   end
      |   if isnan(f32PropGain)
      |     if ~strcmp(f32PropGain_bkup,'0')
      |       set_param(gcb,'f32PropGain','0');
      |     end
      |   else
      |     tmps=num2str(f32PropGain);
      |     if ~strcmp(f32PropGain_bkup,tmps)
      |       set_param(gcb,'f32PropGain',tmps);
      |     end
      |   end
      |   if isnan(f32IntegGain)
      |     if ~strcmp(f32IntegGain_bkup,'0')
      |       set_param(gcb,'f32IntegGain','0');
      |     end
      |   else
      |     tmps=num2str(f32IntegGain);
      |     if ~strcmp(f32IntegGain_bkup,tmps)
      |       set_param(gcb,'f32IntegGain',tmps);
      |     end
      |   end
      |   if isnan(s16PropGainShift)
      |     if ~strcmp(s16PropGainShift_bkup,'0')
      |       set_param(gcb,'s16PropGainShift','0');
      |     end
      |   else
      |     tmps=num2str(s16PropGainShift);
      |     if ~strcmp(s16PropGainShift_bkup,tmps)
      |       set_param(gcb,'s16PropGainShift',tmps);
      |     end
      |   end
      |   if isnan(s16IntegGainShift)
      |     if ~strcmp(s16IntegGainShift_bkup,'0')
      |       set_param(gcb,'s16IntegGainShift','0');
      |     end
      |   else
      |     tmps=num2str(s16IntegGainShift);
      |     if ~strcmp(s16IntegGainShift_bkup,tmps)
      |       set_param(gcb,'s16IntegGainShift',tmps);
      |     end
      |   end
      |   if isnan(f32LowerLimit)
      |     if ~strcmp(f32LowerLimit_bkup,'0')
      |       set_param(gcb,'f32LowerLimit','0');
      |     end
      |   else
      |     tmps=num2str(f32LowerLimit);
      |     if ~strcmp(f32LowerLimit_bkup,tmps)
      |       set_param(gcb,'f32LowerLimit',tmps);
      |     end
      |   end
      |   if isnan(f32UpperLimit)
      |     if ~strcmp(f32UpperLimit_bkup,'0')
      |       set_param(gcb,'f32UpperLimit','0');
      |     end
      |   else
      |     tmps=num2str(f32UpperLimit);
      |     if ~strcmp(f32UpperLimit_bkup,tmps)
      |       set_param(gcb,'f32UpperLimit',tmps);
      |     end
      |   end
      | end
      mask prompts: showStates "Show internal states:"; resetStatesEnable "Internal state after reset:"; showDebugOutputs "Show debugging outputs:"; SampleTime "Sample time (-1 for inherited):"; wf0 "Speed loop natural frequency f0 [Hz]:"; wksi "Speed loop attenuation ξ:"; J "Moment of inertia J [kg*m^2]:"; Kt "Motor torque constant Kt [N*m/A]:"; lambdaFW "Field weakening MA filter smoothing factor λ (0..1):"; Idmax "Maximum negative d-axis current (demagnetization current - CAUTION!) [A]:"; mechspeed "Maximum mechanical speed of the motor [RPM]:"; polepairs "Number of pole pairs of the motor:"; uscale "U_max (maximum DC bus voltage) [V]:"; iscale "I_max (maximum phase current) [A]:"; autoCalcEn "Calculate implementation parameters from physical parameters"; u16NSamples "u16NSamples (GDFLIB_FilterMA - recalculated smoothing factor):"; f32PropGain "f32PropGain (GFLIB_ControllerPIpAW - proportional gain):"; f32IntegGain "f32IntegGain (GFLIB_ControllerPIpAW - integral gain):"; s16PropGainShift "s16PropGainShift (GFLIB_ControllerPIpAW - scaling bitwise shift applied to the proportional gain):"; s16IntegGainShift "s16IntegGainShift (GFLIB_ControllerPIpAW - scaling bitwise shift applied to the integral gain):"; f32LowerLimit "f32LowerLimit (GFLIB_ControllerPIpAW - lower limit):"; f32UpperLimit "f32UpperLimit (GFLIB_ControllerPIpAW - upper limit):"; SampleTime_1 "Discrete sample time:"
      mask help: Field Weakening controller for the PMSM field-oriented control algorithm in 32-bit fixed-point fractional implementation. This block supports re-initialization of the internal state during simulation. If the block is reset, the output of the MA filter and PI controller will be aligned with the inputs f32FilterMAFWOut_preset and f32ControllerPIpAWFWOut_preset. Refer to the AMMCLIB User's Guide for further details.
      mask init:
      | ddName = get_param(bdroot,'DataDictionary');
      | if length(ddName)==0
      |   set_param(bdroot,'DataDictionary','ammclib_types.sldd');
      | else
      |   dd = Simulink.data.dictionary.open(ddName);
      |   data = getSection(dd,'Design Data');
      |   if ~exist(data,'SWLIBS_2Syst_F16')
      |     addDataSource(dd,'ammclib_types.sldd');
      |     saveChanges(dd);
      |   end
      | end
      | 
      | if showStates == 1
      |   % hidden state variables
      |   if strcmp(get_param([gcb '/u16NSamples'], 'BlockType'), 'Inport')
      |     posblk = get_param(gcb, 'Position');
      | 
      |     pos = get_param([gcb, '/u16NSamples'], 'Position');
      |     orient = get_param([gcb, '/u16NSamples'], 'Orientation');
      |     delete_block([gcb, '/u16NSamples']);
      |     add_block('built-in/Ground', [gcb, '/u16NSamples'], 'Position', pos, 'Orientation', orient);
      | 
      |     pos = get_param([gcb, '/f32PropGain'], 'Position');
      |     orient = get_param([gcb, '/f32PropGain'], 'Orientation');
      |     delete_block([gcb, '/f32PropGain']);
      |     add_block('built-in/Ground', [gcb, '/f32PropGain'], 'Position', pos, 'Orientation', orient);
      | 
      |     pos = get_param([gcb, '/f32IntegGain'], 'Position');
      |     orient = get_param([gcb, '/f32IntegGain'], 'Orientation');
      |     delete_block([gcb, '/f32IntegGain']);
      |     add_block('built-in/Ground', [gcb, '/f32IntegGain'], 'Position', pos, 'Orientation', orient);
      | 
      |     pos = get_param([gcb, '/s16PropGainShift'], 'Position');
      |     orient = get_param([gcb, '/s16PropGainShift'], 'Orientation');
      |     delete_block([gcb, '/s16PropGainShift']);
      |     add_block('built-in/Ground', [gcb, '/s16PropGainShift'], 'Position', pos, 'Orientation', orient);
      | 
      |     pos = get_param([gcb, '/s16IntegGainShift'], 'Position');
      |     orient = get_param([gcb, '/s16IntegGainShift'], 'Orientation');
      |     delete_block([gcb, '/s16IntegGainShift']);
      |     add_block('built-in/Ground', [gcb, '/s16IntegGainShift'], 'Position', pos, 'Orientation', orient);
      | 
      |     pos = get_param([gcb, '/f32LowerLimit'], 'Position');
      |     orient = get_param([gcb, '/f32LowerLimit'], 'Orientation');
      |     delete_block([gcb, '/f32LowerLimit']);
      |     add_block('built-in/Ground', [gcb, '/f32LowerLimit'], 'Position', pos, 'Orientation', orient);
      | 
      |     pos = get_param([gcb, '/f32UpperLimit'], 'Position');
      |     orient = get_param([gcb, '/f32UpperLimit'], 'Orientation');
      |     delete_block([gcb, '/f32UpperLimit']);
      |     add_block('built-in/Ground', [gcb, '/f32UpperLimit'], 'Position', pos, 'Orientation', orient);
      | 
      |     pos = get_param([gcb, '/f32IQReqK_1'], 'Position');
      |     orient = get_param([gcb, '/f32IQReqK_1'], 'Orientation');
      |     delete_block([gcb, '/f32IQReqK_1']);
      |     add_block('built-in/Ground', [gcb, '/f32IQReqK_1'], 'Position', pos, 'Orientation', orient);
      | 
      |     pos = get_param([gcb, '/f32Acc'], 'Position');
      |     orient = get_param([gcb, '/f32Acc'], 'Orientation');
      |     delete_block([gcb, '/f32Acc']);
      |     add_block('built-in/Ground', [gcb, '/f32Acc'], 'Position', pos, 'Orientation', orient);
      | 
      |     pos = get_param([gcb, '/f32IntegPartK_1'], 'Position');
      |     orient = get_param([gcb, '/f32IntegPartK_1'], 'Orientation');
      |     delete_block([gcb, '/f32IntegPartK_1']);
      |     add_block('built-in/Ground', [gcb, '/f32IntegPartK_1'], 'Position', pos, 'Orientation', orient);
      | 
      |     pos = get_param([gcb, '/f32InK_1'], 'Position');
      |     orient = get_param([gcb, '/f32InK_1'], 'Orientation');
      |     delete_block([gcb, '/f32InK_1']);
      |     add_block('built-in/Ground', [gcb, '/f32InK_1'], 'Position', pos, 'Orientation', orient);
      | 
      | 
      |     pmask=Simulink.Mask.get(gcb);
      |     pctrl=pmask.getParameter('SampleTime');
      |     pctrl.set('TypeOptions',{'f32IDQReqAmp/SampleTime','f32VelocityFbck/SampleTime','f32IQFbck/SampleTime','f32UQReq/SampleTime','f32UQLim/SampleTime','f32FilterMAFWOut_preset/SampleTime','f32ControllerPIpAWFWOut_preset/SampleTime'});
      | 
      |     pos = get_param([gcb '/f32Acc_Out'], 'Position');
      |     orient = get_param([gcb '/f32Acc_Out'], 'Orientation');
      |     delete_block([gcb '/f32Acc_Out']);
      |     add_block('built-in/Terminator', [gcb '/f32Acc_Out'], 'Position', pos, 'Orientation', orient);
      | 
      |     pos = get_param([gcb '/f32IntegPartK_1_Out'], 'Position');
      |     orient = get_param([gcb '/f32IntegPartK_1_Out'], 'Orientation');
      |     delete_block([gcb '/f32IntegPartK_1_Out']);
      |     add_block('built-in/Terminator', [gcb '/f32IntegPartK_1_Out'], 'Position', pos, 'Orientation', orient);
      | 
      |     pos = get_param([gcb '/f32InK_1_Out'], 'Position');
      |     orient = get_param([gcb '/f32InK_1_Out'], 'Orientation');
      |     delete_block([gcb '/f32InK_1_Out']);
      |     add_block('built-in/Terminator', [gcb '/f32InK_1_Out'], 'Position', pos, 'Orientation', orient);
      | 
      |     if strcmp(get_param([gcb '/f32IQErrSign'], 'BlockType'), 'Outport')
      |       pos = get_param([gcb '/f32IQErrSign'], 'Position');
      |       orient = get_param([gcb '/f32IQErrSign'], 'Orientation');
      |       delete_block([gcb '/f32IQErrSign']);
      |       add_block('built-in/Terminator', [gcb '/f32IQErrSign'], 'Position', pos, 'Orientation', orient);
      | 
      |       pos = get_param([gcb '/f32IQErr'], 'Position');
      |       orient = get_param([gcb '/f32IQErr'], 'Orientation');
      |       delete_block([gcb '/f32IQErr']);
      |       add_block('built-in/Terminator', [gcb '/f32IQErr'], 'Position', pos, 'Orientation', orient);
      | 
      |       pos = get_param([gcb '/f32FWErr'], 'Position');
      |       orient = get_param([gcb '/f32FWErr'], 'Orientation');
      |       delete_block([gcb '/f32FWErr']);
      |       add_block('built-in/Terminator', [gcb '/f32FWErr'], 'Position', pos, 'Orientation', orient);
      | 
      |       pos = get_param([gcb '/f32UQErr'], 'Position');
      |       orient = get_param([gcb '/f32UQErr'], 'Orientation');
      |       delete_block([gcb '/f32UQErr']);
      |       add_block('built-in/Terminator', [gcb '/f32UQErr'], 'Position', pos, 'Orientation', orient);
      | 
      |       pos = get_param([gcb '/f32FWErrFilt'], 'Position');
      |       orient = get_param([gcb '/f32FWErrFilt'], 'Orientation');
      |       delete_block([gcb '/f32FWErrFilt']);
      |       add_block('built-in/Terminator', [gcb '/f32FWErrFilt'], 'Position', pos, 'Orientation', orient);
      | 
      |       pos = get_param([gcb '/f32FWAngle'], 'Position');
      |       orient = get_param([gcb '/f32FWAngle'], 'Orientation');
      |       delete_block([gcb '/f32FWAngle']);
      |       add_block('built-in/Terminator', [gcb '/f32FWAngle'], 'Position', pos, 'Orientation', orient);
      | 
      |       pos = get_param([gcb '/f32FWSin'], 'Position');
      |       orient = get_param([gcb '/f32FWSin'], 'Orientation');
      |       delete_block([gcb '/f32FWSin']);
      |       add_block('built-in/Terminator', [gcb '/f32FWSin'], 'Position', pos, 'Orientation', orient);
      | 
      |       pos = get_param([gcb '/f32FWCos'], 'Position');
      |       orient = get_param([gcb '/f32FWCos'], 'Orientation');
      |       delete_block([gcb '/f32FWCos']);
      |       add_block('built-in/Terminator', [gcb '/f32FWCos'], 'Position', pos, 'Orientation', orient);
      | 
      |     end
      | 
      |     set_param([gcb '/f32IDQReqAmp'], 'Port', '1');
      |     set_param([gcb '/f32VelocityFbck'], 'Port', '2');
      |     set_param([gcb '/f32IQFbck'], 'Port', '3');
      |     set_param([gcb '/f32UQReq'], 'Port', '4');
      |     set_param([gcb '/f32UQLim'], 'Port', '5');
      |     set_param([gcb '/f32FilterMAFWOut_preset'], 'Port', '6');
      |     set_param([gcb '/f32ControllerPIpAWFWOut_preset'], 'Port', '7');
      | 
      |     tmpOutCnt=0;
      |     tmpOutCnt=tmpOutCnt+1;
      |     set_param([gcb '/pIDQReq'], 'Port', num2str(tmpOutCnt));
      |     tmpOutCnt=tmpOutCnt+1;
      |     set_param([gcb '/u16LimitFlag'], 'Port', num2str(tmpOutCnt));
      | 
      |     autoCalcEn=get_param(gcb,'autoCalcEn');
      |     if strcmp(autoCalcEn,'on')
      |       set_param(gcb,'MaskEnables',{'on','on','off','on','on','on','on','on','on','on','on','on','on','on','on','on','on','on','on','on','on','on','off'});
      |     else
      |       set_param(gcb,'MaskEnables',{'on','on','off','on','off','off','off','off','off','off','off','off','off','off','on','on','on','on','on','on','on','on','off'});
      |     end
      | 
      |     if (posblk(4) - posblk(2)) > 200
      |       height = 200;
      |       set_param(gcb,'Position',[posblk(1), posblk(2), posblk(3), posblk(2)+height])
      |     end
      |   end
      | else
      |   % shown state variables
      |   if strcmp(get_param([gcb '/u16NSamples'], 'BlockType'), 'Ground')
      |     posblk = get_param(gcb, 'Position');
      | 
      |     pos = get_param([gcb, '/u16NSamples'], 'Position');
      |     orient = get_param([gcb, '/u16NSamples'], 'Orientation');
      |     delete_block([gcb, '/u16NSamples']);
      |     add_block('built-in/Inport', [gcb, '/u16NSamples'], 'Position', pos, 'Orientation', orient, 'OutDataTypeStr', 'uint16');
      | 
      |     pos = get_param([gcb, '/f32PropGain'], 'Position');
      |     orient = get_param([gcb, '/f32PropGain'], 'Orientation');
      |     delete_block([gcb, '/f32PropGain']);
      |     add_block('built-in/Inport', [gcb, '/f32PropGain'], 'Position', pos, 'Orientation', orient, 'OutDataTypeStr', 'int32');
      | 
      |     pos = get_param([gcb, '/f32IntegGain'], 'Position');
      |     orient = get_param([gcb, '/f32IntegGain'], 'Orientation');
      |     delete_block([gcb, '/f32IntegGain']);
      |     add_block('built-in/Inport', [gcb, '/f32IntegGain'], 'Position', pos, 'Orientation', orient, 'OutDataTypeStr', 'int32');
      | 
      |     pos = get_param([gcb, '/s16PropGainShift'], 'Position');
      |     orient = get_param([gcb, '/s16PropGainShift'], 'Orientation');
      |     delete_block([gcb, '/s16PropGainShift']);
      |     add_block('built-in/Inport', [gcb, '/s16PropGainShift'], 'Position', pos, 'Orientation', orient, 'OutDataTypeStr', 'int16');
      | 
      |     pos = get_param([gcb, '/s16IntegGainShift'], 'Position');
      |     orient = get_param([gcb, '/s16IntegGainShift'], 'Orientation');
      |     delete_block([gcb, '/s16IntegGainShift']);
      |     add_block('built-in/Inport', [gcb, '/s16IntegGainShift'], 'Position', pos, 'Orientation', orient, 'OutDataTypeStr', 'int16');
      | 
      |     pos = get_param([gcb, '/f32LowerLimit'], 'Position');
      |     orient = get_param([gcb, '/f32LowerLimit'], 'Orientation');
      |     delete_block([gcb, '/f32LowerLimit']);
      |     add_block('built-in/Inport', [gcb, '/f32LowerLimit'], 'Position', pos, 'Orientation', orient, 'OutDataTypeStr', 'int32');
      | 
      |     pos = get_param([gcb, '/f32UpperLimit'], 'Position');
      |     orient = get_param([gcb, '/f32UpperLimit'], 'Orientation');
      |     delete_block([gcb, '/f32UpperLimit']);
      |     add_block('built-in/Inport', [gcb, '/f32UpperLimit'], 'Position', pos, 'Orientation', orient, 'OutDataTypeStr', 'int32');
      | 
      |     pos = get_param([gcb, '/f32IQReqK_1'], 'Position');
      |     orient = get_param([gcb, '/f32IQReqK_1'], 'Orientation');
      |     delete_block([gcb, '/f32IQReqK_1']);
      |     add_block('built-in/Inport', [gcb, '/f32IQReqK_1'], 'Position', pos, 'Orientation', orient, 'OutDataTypeStr', 'int32');
      | 
      |     pos = get_param([gcb, '/f32Acc'], 'Position');
      |     orient = get_param([gcb, '/f32Acc'], 'Orientation');
      |     delete_block([gcb, '/f32Acc']);
      |     add_block('built-in/Inport', [gcb, '/f32Acc'], 'Position', pos, 'Orientation', orient, 'OutDataTypeStr', 'int32');
      | 
      |     pos = get_param([gcb, '/f32IntegPartK_1'], 'Position');
      |     orient = get_param([gcb, '/f32IntegPartK_1'], 'Orientation');
      |     delete_block([gcb, '/f32IntegPartK_1']);
      |     add_block('built-in/Inport', [gcb, '/f32IntegPartK_1'], 'Position', pos, 'Orientation', orient, 'OutDataTypeStr', 'int32');
      | 
      |     pos = get_param([gcb, '/f32InK_1'], 'Position');
      |     orient = get_param([gcb, '/f32InK_1'], 'Orientation');
      |     delete_block([gcb, '/f32InK_1']);
      |     add_block('built-in/Inport', [gcb, '/f32InK_1'], 'Position', pos, 'Orientation', orient, 'OutDataTypeStr', 'int32');
      | 
      | 
      | 
      |     pos = get_param([gcb '/f32Acc_Out'], 'Position');
      |     orient = get_param([gcb '/f32Acc_Out'], 'Orientation');
      |     delete_block([gcb '/f32Acc_Out']);
      |     add_block('built-in/Outport', [gcb '/f32Acc_Out'], 'Position', pos, 'Orientation', orient);
      | 
      |     pos = get_param([gcb '/f32IntegPartK_1_Out'], 'Position');
      |     orient = get_param([gcb '/f32IntegPartK_1_Out'], 'Orientation');
      |     delete_block([gcb '/f32IntegPartK_1_Out']);
      |     add_block('built-in/Outport', [gcb '/f32IntegPartK_1_Out'], 'Position', pos, 'Orientation', orient);
      | 
      |     pos = get_param([gcb '/f32InK_1_Out'], 'Position');
      |     orient = get_param([gcb '/f32InK_1_Out'], 'Orientation');
      |     delete_block([gcb '/f32InK_1_Out']);
      |     add_block('built-in/Outport', [gcb '/f32InK_1_Out'], 'Position', pos, 'Orientation', orient);
      | 
      | 
      |     pmask=Simulink.Mask.get(gcb);
      |     pctrl=pmask.getParameter('SampleTime');
      |     pctrl.set('TypeOptions',{'f32IDQReqAmp/SampleTime','f32VelocityFbck/SampleTime','f32IQFbck/SampleTime','f32UQReq/SampleTime','f32UQLim/SampleTime','f32FilterMAFWOut_preset/SampleTime','f32ControllerPIpAWFWOut_preset/SampleTime','u16NSamples/SampleTime','f32PropGain/SampleTime','f32IntegGain/SampleTime','s16PropGainShift/SampleTime','s16IntegGainShift/SampleTime','f32LowerLimit/SampleTime','f32UpperLimit/SampleTime','f32IQReqK_1/SampleTime','f32Acc/SampleTime','f32IntegPartK_1/SampleTime','f32InK_1/SampleTime'});
      | 
      |     if (showDebugOutputs == 2) && (strcmp(get_param([gcb '/f32IQErrSign'], 'BlockType'), 'Terminator'))
      |       pos = get_param([gcb '/f32IQErrSign'], 'Position');
      |       orient = get_param([gcb '/f32IQErrSign'], 'Orientation');
      |       delete_block([gcb '/f32IQErrSign']);
      |       add_block('built-in/Outport', [gcb '/f32IQErrSign'], 'Position', pos, 'Orientation', orient);
      | 
      |       pos = get_param([gcb '/f32IQErr'], 'Position');
      |       orient = get_param([gcb '/f32IQErr'], 'Orientation');
      |       delete_block([gcb '/f32IQErr']);
      |       add_block('built-in/Outport', [gcb '/f32IQErr'], 'Position', pos, 'Orientation', orient);
      | 
      |       pos = get_param([gcb '/f32FWErr'], 'Position');
      |       orient = get_param([gcb '/f32FWErr'], 'Orientation');
      |       delete_block([gcb '/f32FWErr']);
      |       add_block('built-in/Outport', [gcb '/f32FWErr'], 'Position', pos, 'Orientation', orient);
      | 
      |       pos = get_param([gcb '/f32UQErr'], 'Position');
      |       orient = get_param([gcb '/f32UQErr'], 'Orientation');
      |       delete_block([gcb '/f32UQErr']);
      |       add_block('built-in/Outport', [gcb '/f32UQErr'], 'Position', pos, 'Orientation', orient);
      | 
      |       pos = get_param([gcb '/f32FWErrFilt'], 'Position');
      |       orient = get_param([gcb '/f32FWErrFilt'], 'Orientation');
      |       delete_block([gcb '/f32FWErrFilt']);
      |       add_block('built-in/Outport', [gcb '/f32FWErrFilt'], 'Position', pos, 'Orientation', orient);
      | 
      |       pos = get_param([gcb '/f32FWAngle'], 'Position');
      |       orient = get_param([gcb '/f32FWAngle'], 'Orientation');
      |       delete_block([gcb '/f32FWAngle']);
      |       add_block('built-in/Outport', [gcb '/f32FWAngle'], 'Position', pos, 'Orientation', orient);
      | 
      |       pos = get_param([gcb '/f32FWSin'], 'Position');
      |       orient = get_param([gcb '/f32FWSin'], 'Orientation');
      |       delete_block([gcb '/f32FWSin']);
      |       add_block('built-in/Outport', [gcb '/f32FWSin'], 'Position', pos, 'Orientation', orient);
      | 
      |       pos = get_param([gcb '/f32FWCos'], 'Position');
      |       orient = get_param([gcb '/f32FWCos'], 'Orientation');
      |       delete_block([gcb '/f32FWCos']);
      |       add_block('built-in/Outport', [gcb '/f32FWCos'], 'Position', pos, 'Orientation', orient);
      | 
      |     end
      | 
      |     set_param([gcb '/f32IDQReqAmp'], 'Port', '1');
      |     set_param([gcb '/f32VelocityFbck'], 'Port', '2');
      |     set_param([gcb '/f32IQFbck'], 'Port', '3');
      |     set_param([gcb '/f32UQReq'], 'Port', '4');
      |     set_param([gcb '/f32UQLim'], 'Port', '5');
      |     set_param([gcb '/f32FilterMAFWOut_preset'], 'Port', '6');
      |     set_param([gcb '/f32ControllerPIpAWFWOut_preset'], 'Port', '7');
      |     set_param([gcb '/u16NSamples'], 'Port', '8');
      |     set_param([gcb '/f32PropGain'], 'Port', '9');
      |     set_param([gcb '/f32IntegGain'], 'Port', '10');
      |     set_param([gcb '/s16PropGainShift'], 'Port', '11');
      |     set_param([gcb '/s16IntegGainShift'], 'Port', '12');
      |     set_param([gcb '/f32LowerLimit'], 'Port', '13');
      |     set_param([gcb '/f32UpperLimit'], 'Port', '14');
      |     set_param([gcb '/f32IQReqK_1'], 'Port', '15');
      |     set_param([gcb '/f32Acc'], 'Port', '16');
      |     set_param([gcb '/f32IntegPartK_1'], 'Port', '17');
      |     set_param([gcb '/f32InK_1'], 'Port', '18');
      | 
      |     if (showDebugOutputs == 2)
      |       tmpOutCnt=0;
      |       tmpOutCnt=tmpOutCnt+1;
      |       set_param([gcb '/pIDQReq'], 'Port', num2str(tmpOutCnt));
      |       tmpOutCnt=tmpOutCnt+1;
      |       set_param([gcb '/u16LimitFlag'], 'Port', num2str(tmpOutCnt));
      |       tmpOutCnt=tmpOutCnt+1;
      |       set_param([gcb '/f32IQErrSign'], 'Port', num2str(tmpOutCnt));
      |       tmpOutCnt=tmpOutCnt+1;
      |       set_param([gcb '/f32IQErr'], 'Port', num2str(tmpOutCnt));
      |       tmpOutCnt=tmpOutCnt+1;
      |       set_param([gcb '/f32FWErr'], 'Port', num2str(tmpOutCnt));
      |       tmpOutCnt=tmpOutCnt+1;
      |       set_param([gcb '/f32UQErr'], 'Port', num2str(tmpOutCnt));
      |       tmpOutCnt=tmpOutCnt+1;
      |       set_param([gcb '/f32FWErrFilt'], 'Port', num2str(tmpOutCnt));
      |       tmpOutCnt=tmpOutCnt+1;
      |       set_param([gcb '/f32FWAngle'], 'Port', num2str(tmpOutCnt));
      |       tmpOutCnt=tmpOutCnt+1;
      |       set_param([gcb '/f32FWSin'], 'Port', num2str(tmpOutCnt));
      |       tmpOutCnt=tmpOutCnt+1;
      |       set_param([gcb '/f32FWCos'], 'Port', num2str(tmpOutCnt));
      |       tmpOutCnt=tmpOutCnt+1;
      |       set_param([gcb '/f32Acc_Out'], 'Port', num2str(tmpOutCnt));
      |       tmpOutCnt=tmpOutCnt+1;
      |       set_param([gcb '/f32IntegPartK_1_Out'], 'Port', num2str(tmpOutCnt));
      |       tmpOutCnt=tmpOutCnt+1;
      |       set_param([gcb '/f32InK_1_Out'], 'Port', num2str(tmpOutCnt));
      |     else
      |       tmpOutCnt=0;
      |       tmpOutCnt=tmpOutCnt+1;
      |       set_param([gcb '/pIDQReq'], 'Port', num2str(tmpOutCnt));
      |       tmpOutCnt=tmpOutCnt+1;
      |       set_param([gcb '/u16LimitFlag'], 'Port', num2str(tmpOutCnt));
      |       tmpOutCnt=tmpOutCnt+1;
      |       set_param([gcb '/f32Acc_Out'], 'Port', num2str(tmpOutCnt));
      |       tmpOutCnt=tmpOutCnt+1;
      |       set_param([gcb '/f32IntegPartK_1_Out'], 'Port', num2str(tmpOutCnt));
      |       tmpOutCnt=tmpOutCnt+1;
      |       set_param([gcb '/f32InK_1_Out'], 'Port', num2str(tmpOutCnt));
      |     end
      | 
      |     set_param(gcb,'MaskEnables',{'on','on','on','on','off','off','off','off','off','off','off','off','off','off','off','off','off','off','off','off','off','off','off'});
      | 
      |     if (posblk(4) - posblk(2)) < 475
      |       height = 475;
      |       set_param(gcb,'Position',[posblk(1), posblk(2), posblk(3), posblk(2)+height])
      |     end
      |   else
      |     if (showDebugOutputs == 2) && (strcmp(get_param([gcb '/f32IQErrSign'], 'BlockType'), 'Terminator'))
      |       % shown debugging outputs
      |       pos = get_param([gcb '/f32IQErrSign'], 'Position');
      |       orient = get_param([gcb '/f32IQErrSign'], 'Orientation');
      |       delete_block([gcb '/f32IQErrSign']);
      |       add_block('built-in/Outport', [gcb '/f32IQErrSign'], 'Position', pos, 'Orientation', orient);
      | 
      |       pos = get_param([gcb '/f32IQErr'], 'Position');
      |       orient = get_param([gcb '/f32IQErr'], 'Orientation');
      |       delete_block([gcb '/f32IQErr']);
      |       add_block('built-in/Outport', [gcb '/f32IQErr'], 'Position', pos, 'Orientation', orient);
      | 
      |       pos = get_param([gcb '/f32FWErr'], 'Position');
      |       orient = get_param([gcb '/f32FWErr'], 'Orientation');
      |       delete_block([gcb '/f32FWErr']);
      |       add_block('built-in/Outport', [gcb '/f32FWErr'], 'Position', pos, 'Orientation', orient);
      | 
      |       pos = get_param([gcb '/f32UQErr'], 'Position');
      |       orient = get_param([gcb '/f32UQErr'], 'Orientation');
      |       delete_block([gcb '/f32UQErr']);
      |       add_block('built-in/Outport', [gcb '/f32UQErr'], 'Position', pos, 'Orientation', orient);
      | 
      |       pos = get_param([gcb '/f32FWErrFilt'], 'Position');
      |       orient = get_param([gcb '/f32FWErrFilt'], 'Orientation');
      |       delete_block([gcb '/f32FWErrFilt']);
      |       add_block('built-in/Outport', [gcb '/f32FWErrFilt'], 'Position', pos, 'Orientation', orient);
      | 
      |       pos = get_param([gcb '/f32FWAngle'], 'Position');
      |       orient = get_param([gcb '/f32FWAngle'], 'Orientation');
      |       delete_block([gcb '/f32FWAngle']);
      |       add_block('built-in/Outport', [gcb '/f32FWAngle'], 'Position', pos, 'Orientation', orient);
      | 
      |       pos = get_param([gcb '/f32FWSin'], 'Position');
      |       orient = get_param([gcb '/f32FWSin'], 'Orientation');
      |       delete_block([gcb '/f32FWSin']);
      |       add_block('built-in/Outport', [gcb '/f32FWSin'], 'Position', pos, 'Orientation', orient);
      | 
      |       pos = get_param([gcb '/f32FWCos'], 'Position');
      |       orient = get_param([gcb '/f32FWCos'], 'Orientation');
      |       delete_block([gcb '/f32FWCos']);
      |       add_block('built-in/Outport', [gcb '/f32FWCos'], 'Position', pos, 'Orientation', orient);
      | 
      |       tmpOutCnt=0;
      |       tmpOutCnt=tmpOutCnt+1;
      |       set_param([gcb '/pIDQReq'], 'Port', num2str(tmpOutCnt));
      |       tmpOutCnt=tmpOutCnt+1;
      |       set_param([gcb '/u16LimitFlag'], 'Port', num2str(tmpOutCnt));
      |       tmpOutCnt=tmpOutCnt+1;
      |       set_param([gcb '/f32IQErrSign'], 'Port', num2str(tmpOutCnt));
      |       tmpOutCnt=tmpOutCnt+1;
      |       set_param([gcb '/f32IQErr'], 'Port', num2str(tmpOutCnt));
      |       tmpOutCnt=tmpOutCnt+1;
      |       set_param([gcb '/f32FWErr'], 'Port', num2str(tmpOutCnt));
      |       tmpOutCnt=tmpOutCnt+1;
      |       set_param([gcb '/f32UQErr'], 'Port', num2str(tmpOutCnt));
      |       tmpOutCnt=tmpOutCnt+1;
      |       set_param([gcb '/f32FWErrFilt'], 'Port', num2str(tmpOutCnt));
      |       tmpOutCnt=tmpOutCnt+1;
      |       set_param([gcb '/f32FWAngle'], 'Port', num2str(tmpOutCnt));
      |       tmpOutCnt=tmpOutCnt+1;
      |       set_param([gcb '/f32FWSin'], 'Port', num2str(tmpOutCnt));
      |       tmpOutCnt=tmpOutCnt+1;
      |       set_param([gcb '/f32FWCos'], 'Port', num2str(tmpOutCnt));
      |       tmpOutCnt=tmpOutCnt+1;
      |       set_param([gcb '/f32Acc_Out'], 'Port', num2str(tmpOutCnt));
      |       tmpOutCnt=tmpOutCnt+1;
      |       set_param([gcb '/f32IntegPartK_1_Out'], 'Port', num2str(tmpOutCnt));
      |       tmpOutCnt=tmpOutCnt+1;
      |       set_param([gcb '/f32InK_1_Out'], 'Port', num2str(tmpOutCnt));
      |     elseif (showDebugOutputs == 1) && (strcmp(get_param([gcb '/f32IQErrSign'], 'BlockType'), 'Outport'))
      |       % hidden debugging outputs
      |       pos = get_param([gcb '/f32IQErrSign'], 'Position');
      |       orient = get_param([gcb '/f32IQErrSign'], 'Orientation');
      |       delete_block([gcb '/f32IQErrSign']);
      |       add_block('built-in/Terminator', [gcb '/f32IQErrSign'], 'Position', pos, 'Orientation', orient);
      | 
      |       pos = get_param([gcb '/f32IQErr'], 'Position');
      |       orient = get_param([gcb '/f32IQErr'], 'Orientation');
      |       delete_block([gcb '/f32IQErr']);
      |       add_block('built-in/Terminator', [gcb '/f32IQErr'], 'Position', pos, 'Orientation', orient);
      | 
      |       pos = get_param([gcb '/f32FWErr'], 'Position');
      |       orient = get_param([gcb '/f32FWErr'], 'Orientation');
      |       delete_block([gcb '/f32FWErr']);
      |       add_block('built-in/Terminator', [gcb '/f32FWErr'], 'Position', pos, 'Orientation', orient);
      | 
      |       pos = get_param([gcb '/f32UQErr'], 'Position');
      |       orient = get_param([gcb '/f32UQErr'], 'Orientation');
      |       delete_block([gcb '/f32UQErr']);
      |       add_block('built-in/Terminator', [gcb '/f32UQErr'], 'Position', pos, 'Orientation', orient);
      | 
      |       pos = get_param([gcb '/f32FWErrFilt'], 'Position');
      |       orient = get_param([gcb '/f32FWErrFilt'], 'Orientation');
      |       delete_block([gcb '/f32FWErrFilt']);
      |       add_block('built-in/Terminator', [gcb '/f32FWErrFilt'], 'Position', pos, 'Orientation', orient);
      | 
      |       pos = get_param([gcb '/f32FWAngle'], 'Position');
      |       orient = get_param([gcb '/f32FWAngle'], 'Orientation');
      |       delete_block([gcb '/f32FWAngle']);
      |       add_block('built-in/Terminator', [gcb '/f32FWAngle'], 'Position', pos, 'Orientation', orient);
      | 
      |       pos = get_param([gcb '/f32FWSin'], 'Position');
      |       orient = get_param([gcb '/f32FWSin'], 'Orientation');
      |       delete_block([gcb '/f32FWSin']);
      |       add_block('built-in/Terminator', [gcb '/f32FWSin'], 'Position', pos, 'Orientation', orient);
      | 
      |       pos = get_param([gcb '/f32FWCos'], 'Position');
      |       orient = get_param([gcb '/f32FWCos'], 'Orientation');
      |       delete_block([gcb '/f32FWCos']);
      |       add_block('built-in/Terminator', [gcb '/f32FWCos'], 'Position', pos, 'Orientation', orient);
      | 
      |       tmpOutCnt=0;
      |       tmpOutCnt=tmpOutCnt+1;
      |       set_param([gcb '/pIDQReq'], 'Port', num2str(tmpOutCnt));
      |       tmpOutCnt=tmpOutCnt+1;
      |       set_param([gcb '/u16LimitFlag'], 'Port', num2str(tmpOutCnt));
      |       tmpOutCnt=tmpOutCnt+1;
      |       set_param([gcb '/f32Acc_Out'], 'Port', num2str(tmpOutCnt));
      |       tmpOutCnt=tmpOutCnt+1;
      |       set_param([gcb '/f32IntegPartK_1_Out'], 'Port', num2str(tmpOutCnt));
      |       tmpOutCnt=tmpOutCnt+1;
      |       set_param([gcb '/f32InK_1_Out'], 'Port', num2str(tmpOutCnt));
      |     end
      |   end
      | end
      settings: RTWSystemCode=Inline
      mask Help: web([fileparts(which('ammclib_bam_S32K3xx.slx')) '/../doc/S32K3XXMCLUG.pdf'], '-browser')
      mask TypeOptions showStates: Hide (faster execution) | Show (allows debugging; connect feedback loops manually)
      mask Callback showStates:
      | maskStr=get_param(gcb,'showStates');
      | if strcmp(maskStr,'Hide (faster execution)')
      |   if strcmp(get_param([gcb '/u16NSamples'], 'BlockType'), 'Inport')
      |     autoCalcEn=get_param(gcb,'autoCalcEn');
      |     if strcmp(autoCalcEn,'on')
      |       set_param(gcb,'MaskEnables',{'on','on','off','on','on','on','on','on','on','on','on','on','on','on','on','on','on','on','on','on','on','on','off'});
      |     else
      |       set_param(gcb,'MaskEnables',{'on','on','off','on','off','off','off','off','off','off','off','off','off','off','on','on','on','on','on','on','on','on','off'});
      |     end
      |   end
      | else
      |   if strcmp(get_param([gcb '/u16NSamples'], 'BlockType'), 'Ground')
      |     set_param(gcb,'MaskEnables',{'on','on','on','on','off','off','off','off','off','off','off','off','off','off','off','off','off','off','off','off','off','off','off'});
      |   end
      | end
      mask TypeOptions resetStatesEnable: Pre-set according to the first set of inputs after reset | Clear to zero
      mask TypeOptions showDebugOutputs: Hide | Show
      mask TypeOptions SampleTime: f32IDQReqAmp/SampleTime | f32VelocityFbck/SampleTime | f32IQFbck/SampleTime | f32UQReq/SampleTime | f32UQLim/SampleTime | f32FilterMAFWOut_preset/SampleTime | f32ControllerPIpAWFWOut_preset/SampleTime
      mask Callback SampleTime:
      | p=Simulink.Mask.get(gcb);
      | hintText=p.getDialogControl('timeHint');
      | SampleTime=Simulink.data.evalinGlobal(bdroot,get_param(gcb,'SampleTime'));
      | SampleTime_1=str2double(get_param(gcb,'SampleTime_1'));
      | if (((SampleTime==-1) && (~contains(hintText.Prompt,'inherited'))) || ...
      |     ((SampleTime~=-1) && contains(hintText.Prompt,'inherited')) || ...
      |     ((SampleTime~=-1) && (SampleTime_1~=SampleTime)) || ...
      |     ((SampleTime_1~=-1) && contains(hintText.Prompt,'yet')))
      |   if ((SampleTime==-1) && (~contains(hintText.Prompt,'inherited')))
      |     set_param(gcb,'SampleTime_1',num2str(NaN));
      |     SampleTime_1=NaN;
      |   end
      |   if (SampleTime~=-1)
      |     set_param(gcb,'SampleTime_1',num2str(SampleTime));
      |     SampleTime_1=SampleTime;
      |   end
      |   autoCalcEn=get_param(gcb,'autoCalcEn');
      |   if strcmp(autoCalcEn,'on')
      |     p=Simulink.Mask.get(gcb);
      |     hintText=p.getDialogControl('timeHint');
      |     if SampleTime==-1
      |       SampleTime=SampleTime_1;
      |       if isnan(SampleTime)
      |         hintText.Prompt='Note: Implementation parameters cannot be calculated yet because the block''s inherited sample time is unknown. Simulink will update the sample time when you run the simulation.';
      |       else
      |         hintText.Prompt='Caution: Implementation parameters depend on inherited sample time. Make sure that the sample time of the block''s inputs corresponds to the sampling period in the target application.';
      |       end
      |     else
      |       hintText.Prompt='Caution: Implementation parameters depend on the sample time. Make sure that the simulation time step corresponds to the sampling period in the target application.';
      |     end
      |     u16NSamples_bkup=get_param(gcb,'u16NSamples');
      |     f32PropGain_bkup=get_param(gcb,'f32PropGain');
      |     f32IntegGain_bkup=get_param(gcb,'f32IntegGain');
      |     s16PropGainShift_bkup=get_param(gcb,'s16PropGainShift');
      |     s16IntegGainShift_bkup=get_param(gcb,'s16IntegGainShift');
      |     f32LowerLimit_bkup=get_param(gcb,'f32LowerLimit');
      |     f32UpperLimit_bkup=get_param(gcb,'f32UpperLimit');
      |     wf0=Simulink.data.evalinGlobal(bdroot,get_param(gcb,'wf0'));
      |     wksi=Simulink.data.evalinGlobal(bdroot,get_param(gcb,'wksi'));
      |     J=Simulink.data.evalinGlobal(bdroot,get_param(gcb,'J'));
      |     Kt=Simulink.data.evalinGlobal(bdroot,get_param(gcb,'Kt'));
      |     lambdaFW=Simulink.data.evalinGlobal(bdroot,get_param(gcb,'lambdaFW'));
      |     Idmax=Simulink.data.evalinGlobal(bdroot,get_param(gcb,'Idmax'));
      |     mechspeed=Simulink.data.evalinGlobal(bdroot,get_param(gcb,'mechspeed'));
      |     polepairs=Simulink.data.evalinGlobal(bdroot,get_param(gcb,'polepairs'));
      |     uscale=Simulink.data.evalinGlobal(bdroot,get_param(gcb,'uscale'));
      |     iscale=Simulink.data.evalinGlobal(bdroot,get_param(gcb,'iscale'));
      |     if (wf0<=0)
      |       warning('Natural frequency f0 must be positive.');
      |     end
      |     if (wksi<=0)
      |       warning('Current loop attenuation must be positive.');
      |     end
      |     if (wksi>1)
      |       warning('Current loop attenuation must not exceed 1.');
      |     end
      |     if (J<=0)
      |       warning('Moment of inertia J must be positive.');
      |     end
      |     if (Kt<=0)
      |       warning('Torque constant Kt must be positive.');
      |     end
      |     if (lambdaFW<0)
      |       warning('MA filter smoothing factor must be in the range 0..1.');
      |     end
      |     if (lambdaFW>1)
      |       warning('MA filter smoothing factor must be in the range 0..1.');
      |     end
      |     if (mechspeed<=0)
      |       warning('Max. speed must be positive.');
      |     end
      |     if (polepairs<1)
      |       warning('Number of pole pairs must be a natural number (1, 2, 3, ...).');
      |     end
      |     if (round(polepairs)~=polepairs)
      |       warning('Number of pole pairs must be a natural number (1, 2, 3, ...).');
      |     end
      |     if (uscale<=0)
      |       warning('U_max must be positive.');
      |     end
      |     if (iscale<=0)
      |       warning('I_max must be positive.');
      |     end
      |     w0=6.283185307179586*wf0;
      |     pgain=2.0*wksi*w0*J/Kt;
      |     igain=w0*w0*J/Kt;
      |     wmax=polepairs*mechspeed*0.1047197551196598;
      |     kif=igain*SampleTime*0.5*wmax/iscale;
      |     fwkpf=0.9*pgain*wmax/iscale;
      |     s16PropGainShift=ceil(log2(abs(fwkpf)));
      |     if s16PropGainShift<-31
      |       s16PropGainShift=-31;
      |     end
      |     if s16PropGainShift>31
      |       s16PropGainShift=31;
      |       warning(['Parameter s16PropGainShift of ' gcb ' exceeds the fixed-point range.']);
      |     end
      |     f32PropGain=round(fwkpf*2^(-s16PropGainShift)*2^31);
      |     if f32PropGain>2^31-1
      |       f32PropGain=2^31-1;
      |       warning(['Parameter f32PropGain of ' gcb ' exceeds the fixed-point range.']);
      |     end
      |     if f32PropGain<-2^31
      |       f32PropGain=-2^31;
      |       warning(['Parameter f32PropGain of ' gcb ' exceeds the fixed-point range.']);
      |     end
      |     s16IntegGainShift=ceil(log2(abs(kif)));
      |     if s16IntegGainShift<-31
      |       s16IntegGainShift=-31;
      |     end
      |     if s16IntegGainShift>31
      |       s16IntegGainShift=31;
      |       warning(['Parameter s16IntegGainShift of ' gcb ' exceeds the fixed-point range.']);
      |     end
      |     f32IntegGain=round(kif*2^(-s16IntegGainShift)*2^31);
      |     if f32IntegGain>2^31-1
      |       f32IntegGain=2^31-1;
      |       warning(['Parameter f32IntegGain of ' gcb ' exceeds the fixed-point range.']);
      |     end
      |     if f32IntegGain<-2^31
      |       f32IntegGain=-2^31;
      |       warning(['Parameter f32IntegGain of ' gcb ' exceeds the fixed-point range.']);
      |     end
      |     if (Idmax<0)
      |       iratio=abs(Idmax)/iscale;
      |       lowlim=0.3183098861837907*acos(iratio)-0.5;
      |     else
      |       lowlim=0.0;
      |     end
      |     f32LowerLimit=round(lowlim*2^31);
      |     if f32LowerLimit>2^31-1
      |       f32LowerLimit=2^31-1;
      |       warning(['Parameter f32LowerLimit of ' gcb ' exceeds the fixed-point range.']);
      |     end
      |     if f32LowerLimit<-2^31
      |       f32LowerLimit=-2^31;
      |       warning(['Parameter f32LowerLimit of ' gcb ' exceeds the fixed-point range.']);
      |     end
      |     f32UpperLimit=0;
      |     u16NSamples=round(log2(1.0/abs(lambdaFW)));
      |     if u16NSamples>31
      |       u16NSamples=31;
      |     end
      |     if u16NSamples<0
      |       u16NSamples=0;
      |     end
      |     if isnan(u16NSamples)
      |       if ~strcmp(u16NSamples_bkup,'0')
      |         set_param(gcb,'u16NSamples','0');
      |       end
      |     else
      |       tmps=num2str(u16NSamples);
      |       if ~strcmp(u16NSamples_bkup,tmps)
      |         set_param(gcb,'u16NSamples',tmps);
      |       end
      |     end
      |     if isnan(f32PropGain)
      |       if ~strcmp(f32PropGain_bkup,'0')
      |         set_param(gcb,'f32PropGain','0');
      |       end
      |     else
      |       tmps=num2str(f32PropGain);
      |       if ~strcmp(f32PropGain_bkup,tmps)
      |         set_param(gcb,'f32PropGain',tmps);
      |       end
      |     end
      |     if isnan(f32IntegGain)
      |       if ~strcmp(f32IntegGain_bkup,'0')
      |         set_param(gcb,'f32IntegGain','0');
      |       end
      |     else
      |       tmps=num2str(f32IntegGain);
      |       if ~strcmp(f32IntegGain_bkup,tmps)
      |         set_param(gcb,'f32IntegGain',tmps);
      |       end
      |     end
      |     if isnan(s16PropGainShift)
      |       if ~strcmp(s16PropGainShift_bkup,'0')
      |         set_param(gcb,'s16PropGainShift','0');
      |       end
      |     else
      |       tmps=num2str(s16PropGainShift);
      |       if ~strcmp(s16PropGainShift_bkup,tmps)
      |         set_param(gcb,'s16PropGainShift',tmps);
      |       end
      |     end
      |     if isnan(s16IntegGainShift)
      |       if ~strcmp(s16IntegGainShift_bkup,'0')
      |         set_param(gcb,'s16IntegGainShift','0');
      |       end
      |     else
      |       tmps=num2str(s16IntegGainShift);
      |       if ~strcmp(s16IntegGainShift_bkup,tmps)
      |         set_param(gcb,'s16IntegGainShift',tmps);
      |       end
      |     end
      |     if isnan(f32LowerLimit)
      |       if ~strcmp(f32LowerLimit_bkup,'0')
      |         set_param(gcb,'f32LowerLimit','0');
      |       end
      |     else
      |       tmps=num2str(f32LowerLimit);
      |       if ~strcmp(f32LowerLimit_bkup,tmps)
      |         set_param(gcb,'f32LowerLimit',tmps);
      |       end
      |     end
      |     if isnan(f32UpperLimit)
      |       if ~strcmp(f32UpperLimit_bkup,'0')
      |         set_param(gcb,'f32UpperLimit','0');
      |       end
      |     else
      |       tmps=num2str(f32UpperLimit);
      |       if ~strcmp(f32UpperLimit_bkup,tmps)
      |         set_param(gcb,'f32UpperLimit',tmps);
      |       end
      |     end
      |   end
      | end
      mask Callback wf0:
      | autoCalcEn=get_param(gcb,'autoCalcEn');
      | if strcmp(autoCalcEn,'on')
      |   SampleTime=Simulink.data.evalinGlobal(bdroot,get_param(gcb,'SampleTime'));
      |   if (SampleTime==-1)
      |     SampleTime=str2double(get_param(gcb,'SampleTime_1'));
      |   end
      |   u16NSamples_bkup=get_param(gcb,'u16NSamples');
      |   f32PropGain_bkup=get_param(gcb,'f32PropGain');
      |   f32IntegGain_bkup=get_param(gcb,'f32IntegGain');
      |   s16PropGainShift_bkup=get_param(gcb,'s16PropGainShift');
      |   s16IntegGainShift_bkup=get_param(gcb,'s16IntegGainShift');
      |   f32LowerLimit_bkup=get_param(gcb,'f32LowerLimit');
      |   f32UpperLimit_bkup=get_param(gcb,'f32UpperLimit');
      |   wf0=Simulink.data.evalinGlobal(bdroot,get_param(gcb,'wf0'));
      |   wksi=Simulink.data.evalinGlobal(bdroot,get_param(gcb,'wksi'));
      |   J=Simulink.data.evalinGlobal(bdroot,get_param(gcb,'J'));
      |   Kt=Simulink.data.evalinGlobal(bdroot,get_param(gcb,'Kt'));
      |   lambdaFW=Simulink.data.evalinGlobal(bdroot,get_param(gcb,'lambdaFW'));
      |   Idmax=Simulink.data.evalinGlobal(bdroot,get_param(gcb,'Idmax'));
      |   mechspeed=Simulink.data.evalinGlobal(bdroot,get_param(gcb,'mechspeed'));
      |   polepairs=Simulink.data.evalinGlobal(bdroot,get_param(gcb,'polepairs'));
      |   uscale=Simulink.data.evalinGlobal(bdroot,get_param(gcb,'uscale'));
      |   iscale=Simulink.data.evalinGlobal(bdroot,get_param(gcb,'iscale'));
      |   if (wf0<=0)
      |     warning('Natural frequency f0 must be positive.');
      |   end
      |   if (wksi<=0)
      |     warning('Current loop attenuation must be positive.');
      |   end
      |   if (wksi>1)
      |     warning('Current loop attenuation must not exceed 1.');
      |   end
      |   if (J<=0)
      |     warning('Moment of inertia J must be positive.');
      |   end
      |   if (Kt<=0)
      |     warning('Torque constant Kt must be positive.');
      |   end
      |   if (lambdaFW<0)
      |     warning('MA filter smoothing factor must be in the range 0..1.');
      |   end
      |   if (lambdaFW>1)
      |     warning('MA filter smoothing factor must be in the range 0..1.');
      |   end
      |   if (mechspeed<=0)
      |     warning('Max. speed must be positive.');
      |   end
      |   if (polepairs<1)
      |     warning('Number of pole pairs must be a natural number (1, 2, 3, ...).');
      |   end
      |   if (round(polepairs)~=polepairs)
      |     warning('Number of pole pairs must be a natural number (1, 2, 3, ...).');
      |   end
      |   if (uscale<=0)
      |     warning('U_max must be positive.');
      |   end
      |   if (iscale<=0)
      |     warning('I_max must be positive.');
      |   end
      |   w0=6.283185307179586*wf0;
      |   pgain=2.0*wksi*w0*J/Kt;
      |   igain=w0*w0*J/Kt;
      |   wmax=polepairs*mechspeed*0.1047197551196598;
      |   kif=igain*SampleTime*0.5*wmax/iscale;
      |   fwkpf=0.9*pgain*wmax/iscale;
      |   s16PropGainShift=ceil(log2(abs(fwkpf)));
      |   if s16PropGainShift<-31
      |     s16PropGainShift=-31;
      |   end
      |   if s16PropGainShift>31
      |     s16PropGainShift=31;
      |     warning(['Parameter s16PropGainShift of ' gcb ' exceeds the fixed-point range.']);
      |   end
      |   f32PropGain=round(fwkpf*2^(-s16PropGainShift)*2^31);
      |   if f32PropGain>2^31-1
      |     f32PropGain=2^31-1;
      |     warning(['Parameter f32PropGain of ' gcb ' exceeds the fixed-point range.']);
      |   end
      |   if f32PropGain<-2^31
      |     f32PropGain=-2^31;
      |     warning(['Parameter f32PropGain of ' gcb ' exceeds the fixed-point range.']);
      |   end
      |   s16IntegGainShift=ceil(log2(abs(kif)));
      |   if s16IntegGainShift<-31
      |     s16IntegGainShift=-31;
      |   end
      |   if s16IntegGainShift>31
      |     s16IntegGainShift=31;
      |     warning(['Parameter s16IntegGainShift of ' gcb ' exceeds the fixed-point range.']);
      |   end
      |   f32IntegGain=round(kif*2^(-s16IntegGainShift)*2^31);
      |   if f32IntegGain>2^31-1
      |     f32IntegGain=2^31-1;
      |     warning(['Parameter f32IntegGain of ' gcb ' exceeds the fixed-point range.']);
      |   end
      |   if f32IntegGain<-2^31
      |     f32IntegGain=-2^31;
      |     warning(['Parameter f32IntegGain of ' gcb ' exceeds the fixed-point range.']);
      |   end
      |   if (Idmax<0)
      |     iratio=abs(Idmax)/iscale;
      |     lowlim=0.3183098861837907*acos(iratio)-0.5;
      |   else
      |     lowlim=0.0;
      |   end
      |   f32LowerLimit=round(lowlim*2^31);
      |   if f32LowerLimit>2^31-1
      |     f32LowerLimit=2^31-1;
      |     warning(['Parameter f32LowerLimit of ' gcb ' exceeds the fixed-point range.']);
      |   end
      |   if f32LowerLimit<-2^31
      |     f32LowerLimit=-2^31;
      |     warning(['Parameter f32LowerLimit of ' gcb ' exceeds the fixed-point range.']);
      |   end
      |   f32UpperLimit=0;
      |   u16NSamples=round(log2(1.0/abs(lambdaFW)));
      |   if u16NSamples>31
      |     u16NSamples=31;
      |   end
      |   if u16NSamples<0
      |     u16NSamples=0;
      |   end
      |   if isnan(u16NSamples)
      |     if ~strcmp(u16NSamples_bkup,'0')
      |       set_param(gcb,'u16NSamples','0');
      |     end
      |   else
      |     tmps=num2str(u16NSamples);
      |     if ~strcmp(u16NSamples_bkup,tmps)
      |       set_param(gcb,'u16NSamples',tmps);
      |     end
      |   end
      |   if isnan(f32PropGain)
      |     if ~strcmp(f32PropGain_bkup,'0')
      |       set_param(gcb,'f32PropGain','0');
      |     end
      |   else
      |     tmps=num2str(f32PropGain);
      |     if ~strcmp(f32PropGain_bkup,tmps)
      |       set_param(gcb,'f32PropGain',tmps);
      |     end
      |   end
      |   if isnan(f32IntegGain)
      |     if ~strcmp(f32IntegGain_bkup,'0')
      |       set_param(gcb,'f32IntegGain','0');
      |     end
      |   else
      |     tmps=num2str(f32IntegGain);
      |     if ~strcmp(f32IntegGain_bkup,tmps)
      |       set_param(gcb,'f32IntegGain',tmps);
      |     end
      |   end
      |   if isnan(s16PropGainShift)
      |     if ~strcmp(s16PropGainShift_bkup,'0')
      |       set_param(gcb,'s16PropGainShift','0');
      |     end
      |   else
      |     tmps=num2str(s16PropGainShift);
      |     if ~strcmp(s16PropGainShift_bkup,tmps)
      |       set_param(gcb,'s16PropGainShift',tmps);
      |     end
      |   end
      |   if isnan(s16IntegGainShift)
      |     if ~strcmp(s16IntegGainShift_bkup,'0')
      |       set_param(gcb,'s16IntegGainShift','0');
      |     end
      |   else
      |     tmps=num2str(s16IntegGainShift);
      |     if ~strcmp(s16IntegGainShift_bkup,tmps)
      |       set_param(gcb,'s16IntegGainShift',tmps);
      |     end
      |   end
      |   if isnan(f32LowerLimit)
      |     if ~strcmp(f32LowerLimit_bkup,'0')
      |       set_param(gcb,'f32LowerLimit','0');
      |     end
      |   else
      |     tmps=num2str(f32LowerLimit);
      |     if ~strcmp(f32LowerLimit_bkup,tmps)
      |       set_param(gcb,'f32LowerLimit',tmps);
      |     end
      |   end
      |   if isnan(f32UpperLimit)
      |     if ~strcmp(f32UpperLimit_bkup,'0')
      |       set_param(gcb,'f32UpperLimit','0');
      |     end
      |   else
      |     tmps=num2str(f32UpperLimit);
      |     if ~strcmp(f32UpperLimit_bkup,tmps)
      |       set_param(gcb,'f32UpperLimit',tmps);
      |     end
      |   end
      | end
      mask Callback wksi:
      | autoCalcEn=get_param(gcb,'autoCalcEn');
      | if strcmp(autoCalcEn,'on')
      |   SampleTime=Simulink.data.evalinGlobal(bdroot,get_param(gcb,'SampleTime'));
      |   if (SampleTime==-1)
      |     SampleTime=str2double(get_param(gcb,'SampleTime_1'));
      |   end
      |   u16NSamples_bkup=get_param(gcb,'u16NSamples');
      |   f32PropGain_bkup=get_param(gcb,'f32PropGain');
      |   f32IntegGain_bkup=get_param(gcb,'f32IntegGain');
      |   s16PropGainShift_bkup=get_param(gcb,'s16PropGainShift');
      |   s16IntegGainShift_bkup=get_param(gcb,'s16IntegGainShift');
      |   f32LowerLimit_bkup=get_param(gcb,'f32LowerLimit');
      |   f32UpperLimit_bkup=get_param(gcb,'f32UpperLimit');
      |   wf0=Simulink.data.evalinGlobal(bdroot,get_param(gcb,'wf0'));
      |   wksi=Simulink.data.evalinGlobal(bdroot,get_param(gcb,'wksi'));
      |   J=Simulink.data.evalinGlobal(bdroot,get_param(gcb,'J'));
      |   Kt=Simulink.data.evalinGlobal(bdroot,get_param(gcb,'Kt'));
      |   lambdaFW=Simulink.data.evalinGlobal(bdroot,get_param(gcb,'lambdaFW'));
      |   Idmax=Simulink.data.evalinGlobal(bdroot,get_param(gcb,'Idmax'));
      |   mechspeed=Simulink.data.evalinGlobal(bdroot,get_param(gcb,'mechspeed'));
      |   polepairs=Simulink.data.evalinGlobal(bdroot,get_param(gcb,'polepairs'));
      |   uscale=Simulink.data.evalinGlobal(bdroot,get_param(gcb,'uscale'));
      |   iscale=Simulink.data.evalinGlobal(bdroot,get_param(gcb,'iscale'));
      |   if (wf0<=0)
      |     warning('Natural frequency f0 must be positive.');
      |   end
      |   if (wksi<=0)
      |     warning('Current loop attenuation must be positive.');
      |   end
      |   if (wksi>1)
      |     warning('Current loop attenuation must not exceed 1.');
      |   end
      |   if (J<=0)
      |     warning('Moment of inertia J must be positive.');
      |   end
      |   if (Kt<=0)
      |     warning('Torque constant Kt must be positive.');
      |   end
      |   if (lambdaFW<0)
      |     warning('MA filter smoothing factor must be in the range 0..1.');
      |   end
      |   if (lambdaFW>1)
      |     warning('MA filter smoothing factor must be in the range 0..1.');
      |   end
      |   if (mechspeed<=0)
      |     warning('Max. speed must be positive.');
      |   end
      |   if (polepairs<1)
      |     warning('Number of pole pairs must be a natural number (1, 2, 3, ...).');
      |   end
      |   if (round(polepairs)~=polepairs)
      |     warning('Number of pole pairs must be a natural number (1, 2, 3, ...).');
      |   end
      |   if (uscale<=0)
      |     warning('U_max must be positive.');
      |   end
      |   if (iscale<=0)
      |     warning('I_max must be positive.');
      |   end
      |   w0=6.283185307179586*wf0;
      |   pgain=2.0*wksi*w0*J/Kt;
      |   igain=w0*w0*J/Kt;
      |   wmax=polepairs*mechspeed*0.1047197551196598;
      |   kif=igain*SampleTime*0.5*wmax/iscale;
      |   fwkpf=0.9*pgain*wmax/iscale;
      |   s16PropGainShift=ceil(log2(abs(fwkpf)));
      |   if s16PropGainShift<-31
      |     s16PropGainShift=-31;
      |   end
      |   if s16PropGainShift>31
      |     s16PropGainShift=31;
      |     warning(['Parameter s16PropGainShift of ' gcb ' exceeds the fixed-point range.']);
      |   end
      |   f32PropGain=round(fwkpf*2^(-s16PropGainShift)*2^31);
      |   if f32PropGain>2^31-1
      |     f32PropGain=2^31-1;
      |     warning(['Parameter f32PropGain of ' gcb ' exceeds the fixed-point range.']);
      |   end
      |   if f32PropGain<-2^31
      |     f32PropGain=-2^31;
      |     warning(['Parameter f32PropGain of ' gcb ' exceeds the fixed-point range.']);
      |   end
      |   s16IntegGainShift=ceil(log2(abs(kif)));
      |   if s16IntegGainShift<-31
      |     s16IntegGainShift=-31;
      |   end
      |   if s16IntegGainShift>31
      |     s16IntegGainShift=31;
      |     warning(['Parameter s16IntegGainShift of ' gcb ' exceeds the fixed-point range.']);
      |   end
      |   f32IntegGain=round(kif*2^(-s16IntegGainShift)*2^31);
      |   if f32IntegGain>2^31-1
      |     f32IntegGain=2^31-1;
      |     warning(['Parameter f32IntegGain of ' gcb ' exceeds the fixed-point range.']);
      |   end
      |   if f32IntegGain<-2^31
      |     f32IntegGain=-2^31;
      |     warning(['Parameter f32IntegGain of ' gcb ' exceeds the fixed-point range.']);
      |   end
      |   if (Idmax<0)
      |     iratio=abs(Idmax)/iscale;
      |     lowlim=0.3183098861837907*acos(iratio)-0.5;
      |   else
      |     lowlim=0.0;
      |   end
      |   f32LowerLimit=round(lowlim*2^31);
      |   if f32LowerLimit>2^31-1
      |     f32LowerLimit=2^31-1;
      |     warning(['Parameter f32LowerLimit of ' gcb ' exceeds the fixed-point range.']);
      |   end
      |   if f32LowerLimit<-2^31
      |     f32LowerLimit=-2^31;
      |     warning(['Parameter f32LowerLimit of ' gcb ' exceeds the fixed-point range.']);
      |   end
      |   f32UpperLimit=0;
      |   u16NSamples=round(log2(1.0/abs(lambdaFW)));
      |   if u16NSamples>31
      |     u16NSamples=31;
      |   end
      |   if u16NSamples<0
      |     u16NSamples=0;
      |   end
      |   if isnan(u16NSamples)
      |     if ~strcmp(u16NSamples_bkup,'0')
      |       set_param(gcb,'u16NSamples','0');
      |     end
      |   else
      |     tmps=num2str(u16NSamples);
      |     if ~strcmp(u16NSamples_bkup,tmps)
      |       set_param(gcb,'u16NSamples',tmps);
      |     end
      |   end
      |   if isnan(f32PropGain)
      |     if ~strcmp(f32PropGain_bkup,'0')
      |       set_param(gcb,'f32PropGain','0');
      |     end
      |   else
      |     tmps=num2str(f32PropGain);
      |     if ~strcmp(f32PropGain_bkup,tmps)
      |       set_param(gcb,'f32PropGain',tmps);
      |     end
      |   end
      |   if isnan(f32IntegGain)
      |     if ~strcmp(f32IntegGain_bkup,'0')
      |       set_param(gcb,'f32IntegGain','0');
      |     end
      |   else
      |     tmps=num2str(f32IntegGain);
      |     if ~strcmp(f32IntegGain_bkup,tmps)
      |       set_param(gcb,'f32IntegGain',tmps);
      |     end
      |   end
      |   if isnan(s16PropGainShift)
      |     if ~strcmp(s16PropGainShift_bkup,'0')
      |       set_param(gcb,'s16PropGainShift','0');
      |     end
      |   else
      |     tmps=num2str(s16PropGainShift);
      |     if ~strcmp(s16PropGainShift_bkup,tmps)
      |       set_param(gcb,'s16PropGainShift',tmps);
      |     end
      |   end
      |   if isnan(s16IntegGainShift)
      |     if ~strcmp(s16IntegGainShift_bkup,'0')
      |       set_param(gcb,'s16IntegGainShift','0');
      |     end
      |   else
      |     tmps=num2str(s16IntegGainShift);
      |     if ~strcmp(s16IntegGainShift_bkup,tmps)
      |       set_param(gcb,'s16IntegGainShift',tmps);
      |     end
      |   end
      |   if isnan(f32LowerLimit)
      |     if ~strcmp(f32LowerLimit_bkup,'0')
      |       set_param(gcb,'f32LowerLimit','0');
      |     end
      |   else
      |     tmps=num2str(f32LowerLimit);
      |     if ~strcmp(f32LowerLimit_bkup,tmps)
      |       set_param(gcb,'f32LowerLimit',tmps);
      |     end
      |   end
      |   if isnan(f32UpperLimit)
      |     if ~strcmp(f32UpperLimit_bkup,'0')
      |       set_param(gcb,'f32UpperLimit','0');
      |     end
      |   else
      |     tmps=num2str(f32UpperLimit);
      |     if ~strcmp(f32UpperLimit_bkup,tmps)
      |       set_param(gcb,'f32UpperLimit',tmps);
      |     end
      |   end
      | end
      mask Callback J:
      | autoCalcEn=get_param(gcb,'autoCalcEn');
      | if strcmp(autoCalcEn,'on')
      |   SampleTime=Simulink.data.evalinGlobal(bdroot,get_param(gcb,'SampleTime'));
      |   if (SampleTime==-1)
      |     SampleTime=str2double(get_param(gcb,'SampleTime_1'));
      |   end
      |   u16NSamples_bkup=get_param(gcb,'u16NSamples');
      |   f32PropGain_bkup=get_param(gcb,'f32PropGain');
      |   f32IntegGain_bkup=get_param(gcb,'f32IntegGain');
      |   s16PropGainShift_bkup=get_param(gcb,'s16PropGainShift');
      |   s16IntegGainShift_bkup=get_param(gcb,'s16IntegGainShift');
      |   f32LowerLimit_bkup=get_param(gcb,'f32LowerLimit');
      |   f32UpperLimit_bkup=get_param(gcb,'f32UpperLimit');
      |   wf0=Simulink.data.evalinGlobal(bdroot,get_param(gcb,'wf0'));
      |   wksi=Simulink.data.evalinGlobal(bdroot,get_param(gcb,'wksi'));
      |   J=Simulink.data.evalinGlobal(bdroot,get_param(gcb,'J'));
      |   Kt=Simulink.data.evalinGlobal(bdroot,get_param(gcb,'Kt'));
      |   lambdaFW=Simulink.data.evalinGlobal(bdroot,get_param(gcb,'lambdaFW'));
      |   Idmax=Simulink.data.evalinGlobal(bdroot,get_param(gcb,'Idmax'));
      |   mechspeed=Simulink.data.evalinGlobal(bdroot,get_param(gcb,'mechspeed'));
      |   polepairs=Simulink.data.evalinGlobal(bdroot,get_param(gcb,'polepairs'));
      |   uscale=Simulink.data.evalinGlobal(bdroot,get_param(gcb,'uscale'));
      |   iscale=Simulink.data.evalinGlobal(bdroot,get_param(gcb,'iscale'));
      |   if (wf0<=0)
      |     warning('Natural frequency f0 must be positive.');
      |   end
      |   if (wksi<=0)
      |     warning('Current loop attenuation must be positive.');
      |   end
      |   if (wksi>1)
      |     warning('Current loop attenuation must not exceed 1.');
      |   end
      |   if (J<=0)
      |     warning('Moment of inertia J must be positive.');
      |   end
      |   if (Kt<=0)
      |     warning('Torque constant Kt must be positive.');
      |   end
      |   if (lambdaFW<0)
      |     warning('MA filter smoothing factor must be in the range 0..1.');
      |   end
      |   if (lambdaFW>1)
      |     warning('MA filter smoothing factor must be in the range 0..1.');
      |   end
      |   if (mechspeed<=0)
      |     warning('Max. speed must be positive.');
      |   end
      |   if (polepairs<1)
      |     warning('Number of pole pairs must be a natural number (1, 2, 3, ...).');
      |   end
      |   if (round(polepairs)~=polepairs)
      |     warning('Number of pole pairs must be a natural number (1, 2, 3, ...).');
      |   end
      |   if (uscale<=0)
      |     warning('U_max must be positive.');
      |   end
      |   if (iscale<=0)
      |     warning('I_max must be positive.');
      |   end
      |   w0=6.283185307179586*wf0;
      |   pgain=2.0*wksi*w0*J/Kt;
      |   igain=w0*w0*J/Kt;
      |   wmax=polepairs*mechspeed*0.1047197551196598;
      |   kif=igain*SampleTime*0.5*wmax/iscale;
      |   fwkpf=0.9*pgain*wmax/iscale;
      |   s16PropGainShift=ceil(log2(abs(fwkpf)));
      |   if s16PropGainShift<-31
      |     s16PropGainShift=-31;
      |   end
      |   if s16PropGainShift>31
      |     s16PropGainShift=31;
      |     warning(['Parameter s16PropGainShift of ' gcb ' exceeds the fixed-point range.']);
      |   end
      |   f32PropGain=round(fwkpf*2^(-s16PropGainShift)*2^31);
      |   if f32PropGain>2^31-1
      |     f32PropGain=2^31-1;
      |     warning(['Parameter f32PropGain of ' gcb ' exceeds the fixed-point range.']);
      |   end
      |   if f32PropGain<-2^31
      |     f32PropGain=-2^31;
      |     warning(['Parameter f32PropGain of ' gcb ' exceeds the fixed-point range.']);
      |   end
      |   s16IntegGainShift=ceil(log2(abs(kif)));
      |   if s16IntegGainShift<-31
      |     s16IntegGainShift=-31;
      |   end
      |   if s16IntegGainShift>31
      |     s16IntegGainShift=31;
      |     warning(['Parameter s16IntegGainShift of ' gcb ' exceeds the fixed-point range.']);
      |   end
      |   f32IntegGain=round(kif*2^(-s16IntegGainShift)*2^31);
      |   if f32IntegGain>2^31-1
      |     f32IntegGain=2^31-1;
      |     warning(['Parameter f32IntegGain of ' gcb ' exceeds the fixed-point range.']);
      |   end
      |   if f32IntegGain<-2^31
      |     f32IntegGain=-2^31;
      |     warning(['Parameter f32IntegGain of ' gcb ' exceeds the fixed-point range.']);
      |   end
      |   if (Idmax<0)
      |     iratio=abs(Idmax)/iscale;
      |     lowlim=0.3183098861837907*acos(iratio)-0.5;
      |   else
      |     lowlim=0.0;
      |   end
      |   f32LowerLimit=round(lowlim*2^31);
      |   if f32LowerLimit>2^31-1
      |     f32LowerLimit=2^31-1;
      |     warning(['Parameter f32LowerLimit of ' gcb ' exceeds the fixed-point range.']);
      |   end
      |   if f32LowerLimit<-2^31
      |     f32LowerLimit=-2^31;
      |     warning(['Parameter f32LowerLimit of ' gcb ' exceeds the fixed-point range.']);
      |   end
      |   f32UpperLimit=0;
      |   u16NSamples=round(log2(1.0/abs(lambdaFW)));
      |   if u16NSamples>31
      |     u16NSamples=31;
      |   end
      |   if u16NSamples<0
      |     u16NSamples=0;
      |   end
      |   if isnan(u16NSamples)
      |     if ~strcmp(u16NSamples_bkup,'0')
      |       set_param(gcb,'u16NSamples','0');
      |     end
      |   else
      |     tmps=num2str(u16NSamples);
      |     if ~strcmp(u16NSamples_bkup,tmps)
      |       set_param(gcb,'u16NSamples',tmps);
      |     end
      |   end
      |   if isnan(f32PropGain)
      |     if ~strcmp(f32PropGain_bkup,'0')
      |       set_param(gcb,'f32PropGain','0');
      |     end
      |   else
      |     tmps=num2str(f32PropGain);
      |     if ~strcmp(f32PropGain_bkup,tmps)
      |       set_param(gcb,'f32PropGain',tmps);
      |     end
      |   end
      |   if isnan(f32IntegGain)
      |     if ~strcmp(f32IntegGain_bkup,'0')
      |       set_param(gcb,'f32IntegGain','0');
      |     end
      |   else
      |     tmps=num2str(f32IntegGain);
      |     if ~strcmp(f32IntegGain_bkup,tmps)
      |       set_param(gcb,'f32IntegGain',tmps);
      |     end
      |   end
      |   if isnan(s16PropGainShift)
      |     if ~strcmp(s16PropGainShift_bkup,'0')
      |       set_param(gcb,'s16PropGainShift','0');
      |     end
      |   else
      |     tmps=num2str(s16PropGainShift);
      |     if ~strcmp(s16PropGainShift_bkup,tmps)
      |       set_param(gcb,'s16PropGainShift',tmps);
      |     end
      |   end
      |   if isnan(s16IntegGainShift)
      |     if ~strcmp(s16IntegGainShift_bkup,'0')
      |       set_param(gcb,'s16IntegGainShift','0');
      |     end
      |   else
      |     tmps=num2str(s16IntegGainShift);
      |     if ~strcmp(s16IntegGainShift_bkup,tmps)
      |       set_param(gcb,'s16IntegGainShift',tmps);
      |     end
      |   end
      |   if isnan(f32LowerLimit)
      |     if ~strcmp(f32LowerLimit_bkup,'0')
      |       set_param(gcb,'f32LowerLimit','0');
      |     end
      |   else
      |     tmps=num2str(f32LowerLimit);
      |     if ~strcmp(f32LowerLimit_bkup,tmps)
      |       set_param(gcb,'f32LowerLimit',tmps);
      |     end
      |   end
      |   if isnan(f32UpperLimit)
      |     if ~strcmp(f32UpperLimit_bkup,'0')
      |       set_param(gcb,'f32UpperLimit','0');
      |     end
      |   else
      |     tmps=num2str(f32UpperLimit);
      |     if ~strcmp(f32UpperLimit_bkup,tmps)
      |       set_param(gcb,'f32UpperLimit',tmps);
      |     end
      |   end
      | end
      mask Callback Kt:
      | autoCalcEn=get_param(gcb,'autoCalcEn');
      | if strcmp(autoCalcEn,'on')
      |   SampleTime=Simulink.data.evalinGlobal(bdroot,get_param(gcb,'SampleTime'));
      |   if (SampleTime==-1)
      |     SampleTime=str2double(get_param(gcb,'SampleTime_1'));
      |   end
      |   u16NSamples_bkup=get_param(gcb,'u16NSamples');
      |   f32PropGain_bkup=get_param(gcb,'f32PropGain');
      |   f32IntegGain_bkup=get_param(gcb,'f32IntegGain');
      |   s16PropGainShift_bkup=get_param(gcb,'s16PropGainShift');
      |   s16IntegGainShift_bkup=get_param(gcb,'s16IntegGainShift');
      |   f32LowerLimit_bkup=get_param(gcb,'f32LowerLimit');
      |   f32UpperLimit_bkup=get_param(gcb,'f32UpperLimit');
      |   wf0=Simulink.data.evalinGlobal(bdroot,get_param(gcb,'wf0'));
      |   wksi=Simulink.data.evalinGlobal(bdroot,get_param(gcb,'wksi'));
      |   J=Simulink.data.evalinGlobal(bdroot,get_param(gcb,'J'));
      |   Kt=Simulink.data.evalinGlobal(bdroot,get_param(gcb,'Kt'));
      |   lambdaFW=Simulink.data.evalinGlobal(bdroot,get_param(gcb,'lambdaFW'));
      |   Idmax=Simulink.data.evalinGlobal(bdroot,get_param(gcb,'Idmax'));
      |   mechspeed=Simulink.data.evalinGlobal(bdroot,get_param(gcb,'mechspeed'));
      |   polepairs=Simulink.data.evalinGlobal(bdroot,get_param(gcb,'polepairs'));
      |   uscale=Simulink.data.evalinGlobal(bdroot,get_param(gcb,'uscale'));
      |   iscale=Simulink.data.evalinGlobal(bdroot,get_param(gcb,'iscale'));
      |   if (wf0<=0)
      |     warning('Natural frequency f0 must be positive.');
      |   end
      |   if (wksi<=0)
      |     warning('Current loop attenuation must be positive.');
      |   end
      |   if (wksi>1)
      |     warning('Current loop attenuation must not exceed 1.');
      |   end
      |   if (J<=0)
      |     warning('Moment of inertia J must be positive.');
      |   end
      |   if (Kt<=0)
      |     warning('Torque constant Kt must be positive.');
      |   end
      |   if (lambdaFW<0)
      |     warning('MA filter smoothing factor must be in the range 0..1.');
      |   end
      |   if (lambdaFW>1)
      |     warning('MA filter smoothing factor must be in the range 0..1.');
      |   end
      |   if (mechspeed<=0)
      |     warning('Max. speed must be positive.');
      |   end
      |   if (polepairs<1)
      |     warning('Number of pole pairs must be a natural number (1, 2, 3, ...).');
      |   end
      |   if (round(polepairs)~=polepairs)
      |     warning('Number of pole pairs must be a natural number (1, 2, 3, ...).');
      |   end
      |   if (uscale<=0)
      |     warning('U_max must be positive.');
      |   end
      |   if (iscale<=0)
      |     warning('I_max must be positive.');
      |   end
      |   w0=6.283185307179586*wf0;
      |   pgain=2.0*wksi*w0*J/Kt;
      |   igain=w0*w0*J/Kt;
      |   wmax=polepairs*mechspeed*0.1047197551196598;
      |   kif=igain*SampleTime*0.5*wmax/iscale;
      |   fwkpf=0.9*pgain*wmax/iscale;
      |   s16PropGainShift=ceil(log2(abs(fwkpf)));
      |   if s16PropGainShift<-31
      |     s16PropGainShift=-31;
      |   end
      |   if s16PropGainShift>31
      |     s16PropGainShift=31;
      |     warning(['Parameter s16PropGainShift of ' gcb ' exceeds the fixed-point range.']);
      |   end
      |   f32PropGain=round(fwkpf*2^(-s16PropGainShift)*2^31);
      |   if f32PropGain>2^31-1
      |     f32PropGain=2^31-1;
      |     warning(['Parameter f32PropGain of ' gcb ' exceeds the fixed-point range.']);
      |   end
      |   if f32PropGain<-2^31
      |     f32PropGain=-2^31;
      |     warning(['Parameter f32PropGain of ' gcb ' exceeds the fixed-point range.']);
      |   end
      |   s16IntegGainShift=ceil(log2(abs(kif)));
      |   if s16IntegGainShift<-31
      |     s16IntegGainShift=-31;
      |   end
      |   if s16IntegGainShift>31
      |     s16IntegGainShift=31;
      |     warning(['Parameter s16IntegGainShift of ' gcb ' exceeds the fixed-point range.']);
      |   end
      |   f32IntegGain=round(kif*2^(-s16IntegGainShift)*2^31);
      |   if f32IntegGain>2^31-1
      |     f32IntegGain=2^31-1;
      |     warning(['Parameter f32IntegGain of ' gcb ' exceeds the fixed-point range.']);
      |   end
      |   if f32IntegGain<-2^31
      |     f32IntegGain=-2^31;
      |     warning(['Parameter f32IntegGain of ' gcb ' exceeds the fixed-point range.']);
      |   end
      |   if (Idmax<0)
      |     iratio=abs(Idmax)/iscale;
      |     lowlim=0.3183098861837907*acos(iratio)-0.5;
      |   else
      |     lowlim=0.0;
      |   end
      |   f32LowerLimit=round(lowlim*2^31);
      |   if f32LowerLimit>2^31-1
      |     f32LowerLimit=2^31-1;
      |     warning(['Parameter f32LowerLimit of ' gcb ' exceeds the fixed-point range.']);
      |   end
      |   if f32LowerLimit<-2^31
      |     f32LowerLimit=-2^31;
      |     warning(['Parameter f32LowerLimit of ' gcb ' exceeds the fixed-point range.']);
      |   end
      |   f32UpperLimit=0;
      |   u16NSamples=round(log2(1.0/abs(lambdaFW)));
      |   if u16NSamples>31
      |     u16NSamples=31;
      |   end
      |   if u16NSamples<0
      |     u16NSamples=0;
      |   end
      |   if isnan(u16NSamples)
      |     if ~strcmp(u16NSamples_bkup,'0')
      |       set_param(gcb,'u16NSamples','0');
      |     end
      |   else
      |     tmps=num2str(u16NSamples);
      |     if ~strcmp(u16NSamples_bkup,tmps)
      |       set_param(gcb,'u16NSamples',tmps);
      |     end
      |   end
      |   if isnan(f32PropGain)
      |     if ~strcmp(f32PropGain_bkup,'0')
      |       set_param(gcb,'f32PropGain','0');
      |     end
      |   else
      |     tmps=num2str(f32PropGain);
      |     if ~strcmp(f32PropGain_bkup,tmps)
      |       set_param(gcb,'f32PropGain',tmps);
      |     end
      |   end
      |   if isnan(f32IntegGain)
      |     if ~strcmp(f32IntegGain_bkup,'0')
      |       set_param(gcb,'f32IntegGain','0');
      |     end
      |   else
      |     tmps=num2str(f32IntegGain);
      |     if ~strcmp(f32IntegGain_bkup,tmps)
      |       set_param(gcb,'f32IntegGain',tmps);
      |     end
      |   end
      |   if isnan(s16PropGainShift)
      |     if ~strcmp(s16PropGainShift_bkup,'0')
      |       set_param(gcb,'s16PropGainShift','0');
      |     end
      |   else
      |     tmps=num2str(s16PropGainShift);
      |     if ~strcmp(s16PropGainShift_bkup,tmps)
      |       set_param(gcb,'s16PropGainShift',tmps);
      |     end
      |   end
      |   if isnan(s16IntegGainShift)
      |     if ~strcmp(s16IntegGainShift_bkup,'0')
      |       set_param(gcb,'s16IntegGainShift','0');
      |     end
      |   else
      |     tmps=num2str(s16IntegGainShift);
      |     if ~strcmp(s16IntegGainShift_bkup,tmps)
      |       set_param(gcb,'s16IntegGainShift',tmps);
      |     end
      |   end
      |   if isnan(f32LowerLimit)
      |     if ~strcmp(f32LowerLimit_bkup,'0')
      |       set_param(gcb,'f32LowerLimit','0');
      |     end
      |   else
      |     tmps=num2str(f32LowerLimit);
      |     if ~strcmp(f32LowerLimit_bkup,tmps)
      |       set_param(gcb,'f32LowerLimit',tmps);
      |     end
      |   end
      |   if isnan(f32UpperLimit)
      |     if ~strcmp(f32UpperLimit_bkup,'0')
      |       set_param(gcb,'f32UpperLimit','0');
      |     end
      |   else
      |     tmps=num2str(f32UpperLimit);
      |     if ~strcmp(f32UpperLimit_bkup,tmps)
      |       set_param(gcb,'f32UpperLimit',tmps);
      |     end
      |   end
      | end
      mask Callback lambdaFW:
      | autoCalcEn=get_param(gcb,'autoCalcEn');
      | if strcmp(autoCalcEn,'on')
      |   SampleTime=Simulink.data.evalinGlobal(bdroot,get_param(gcb,'SampleTime'));
      |   if (SampleTime==-1)
      |     SampleTime=str2double(get_param(gcb,'SampleTime_1'));
      |   end
      |   u16NSamples_bkup=get_param(gcb,'u16NSamples');
      |   f32PropGain_bkup=get_param(gcb,'f32PropGain');
      |   f32IntegGain_bkup=get_param(gcb,'f32IntegGain');
      |   s16PropGainShift_bkup=get_param(gcb,'s16PropGainShift');
      |   s16IntegGainShift_bkup=get_param(gcb,'s16IntegGainShift');
      |   f32LowerLimit_bkup=get_param(gcb,'f32LowerLimit');
      |   f32UpperLimit_bkup=get_param(gcb,'f32UpperLimit');
      |   wf0=Simulink.data.evalinGlobal(bdroot,get_param(gcb,'wf0'));
      |   wksi=Simulink.data.evalinGlobal(bdroot,get_param(gcb,'wksi'));
      |   J=Simulink.data.evalinGlobal(bdroot,get_param(gcb,'J'));
      |   Kt=Simulink.data.evalinGlobal(bdroot,get_param(gcb,'Kt'));
      |   lambdaFW=Simulink.data.evalinGlobal(bdroot,get_param(gcb,'lambdaFW'));
      |   Idmax=Simulink.data.evalinGlobal(bdroot,get_param(gcb,'Idmax'));
      |   mechspeed=Simulink.data.evalinGlobal(bdroot,get_param(gcb,'mechspeed'));
      |   polepairs=Simulink.data.evalinGlobal(bdroot,get_param(gcb,'polepairs'));
      |   uscale=Simulink.data.evalinGlobal(bdroot,get_param(gcb,'uscale'));
      |   iscale=Simulink.data.evalinGlobal(bdroot,get_param(gcb,'iscale'));
      |   if (wf0<=0)
      |     warning('Natural frequency f0 must be positive.');
      |   end
      |   if (wksi<=0)
      |     warning('Current loop attenuation must be positive.');
      |   end
      |   if (wksi>1)
      |     warning('Current loop attenuation must not exceed 1.');
      |   end
      |   if (J<=0)
      |     warning('Moment of inertia J must be positive.');
      |   end
      |   if (Kt<=0)
      |     warning('Torque constant Kt must be positive.');
      |   end
      |   if (lambdaFW<0)
      |     warning('MA filter smoothing factor must be in the range 0..1.');
      |   end
      |   if (lambdaFW>1)
      |     warning('MA filter smoothing factor must be in the range 0..1.');
      |   end
      |   if (mechspeed<=0)
      |     warning('Max. speed must be positive.');
      |   end
      |   if (polepairs<1)
      |     warning('Number of pole pairs must be a natural number (1, 2, 3, ...).');
      |   end
      |   if (round(polepairs)~=polepairs)
      |     warning('Number of pole pairs must be a natural number (1, 2, 3, ...).');
      |   end
      |   if (uscale<=0)
      |     warning('U_max must be positive.');
      |   end
      |   if (iscale<=0)
      |     warning('I_max must be positive.');
      |   end
      |   w0=6.283185307179586*wf0;
      |   pgain=2.0*wksi*w0*J/Kt;
      |   igain=w0*w0*J/Kt;
      |   wmax=polepairs*mechspeed*0.1047197551196598;
      |   kif=igain*SampleTime*0.5*wmax/iscale;
      |   fwkpf=0.9*pgain*wmax/iscale;
      |   s16PropGainShift=ceil(log2(abs(fwkpf)));
      |   if s16PropGainShift<-31
      |     s16PropGainShift=-31;
      |   end
      |   if s16PropGainShift>31
      |     s16PropGainShift=31;
      |     warning(['Parameter s16PropGainShift of ' gcb ' exceeds the fixed-point range.']);
      |   end
      |   f32PropGain=round(fwkpf*2^(-s16PropGainShift)*2^31);
      |   if f32PropGain>2^31-1
      |     f32PropGain=2^31-1;
      |     warning(['Parameter f32PropGain of ' gcb ' exceeds the fixed-point range.']);
      |   end
      |   if f32PropGain<-2^31
      |     f32PropGain=-2^31;
      |     warning(['Parameter f32PropGain of ' gcb ' exceeds the fixed-point range.']);
      |   end
      |   s16IntegGainShift=ceil(log2(abs(kif)));
      |   if s16IntegGainShift<-31
      |     s16IntegGainShift=-31;
      |   end
      |   if s16IntegGainShift>31
      |     s16IntegGainShift=31;
      |     warning(['Parameter s16IntegGainShift of ' gcb ' exceeds the fixed-point range.']);
      |   end
      |   f32IntegGain=round(kif*2^(-s16IntegGainShift)*2^31);
      |   if f32IntegGain>2^31-1
      |     f32IntegGain=2^31-1;
      |     warning(['Parameter f32IntegGain of ' gcb ' exceeds the fixed-point range.']);
      |   end
      |   if f32IntegGain<-2^31
      |     f32IntegGain=-2^31;
      |     warning(['Parameter f32IntegGain of ' gcb ' exceeds the fixed-point range.']);
      |   end
      |   if (Idmax<0)
      |     iratio=abs(Idmax)/iscale;
      |     lowlim=0.3183098861837907*acos(iratio)-0.5;
      |   else
      |     lowlim=0.0;
      |   end
      |   f32LowerLimit=round(lowlim*2^31);
      |   if f32LowerLimit>2^31-1
      |     f32LowerLimit=2^31-1;
      |     warning(['Parameter f32LowerLimit of ' gcb ' exceeds the fixed-point range.']);
      |   end
      |   if f32LowerLimit<-2^31
      |     f32LowerLimit=-2^31;
      |     warning(['Parameter f32LowerLimit of ' gcb ' exceeds the fixed-point range.']);
      |   end
      |   f32UpperLimit=0;
      |   u16NSamples=round(log2(1.0/abs(lambdaFW)));
      |   if u16NSamples>31
      |     u16NSamples=31;
      |   end
      |   if u16NSamples<0
      |     u16NSamples=0;
      |   end
      |   if isnan(u16NSamples)
      |     if ~strcmp(u16NSamples_bkup,'0')
      |       set_param(gcb,'u16NSamples','0');
      |     end
      |   else
      |     tmps=num2str(u16NSamples);
      |     if ~strcmp(u16NSamples_bkup,tmps)
      |       set_param(gcb,'u16NSamples',tmps);
      |     end
      |   end
      |   if isnan(f32PropGain)
      |     if ~strcmp(f32PropGain_bkup,'0')
      |       set_param(gcb,'f32PropGain','0');
      |     end
      |   else
      |     tmps=num2str(f32PropGain);
      |     if ~strcmp(f32PropGain_bkup,tmps)
      |       set_param(gcb,'f32PropGain',tmps);
      |     end
      |   end
      |   if isnan(f32IntegGain)
      |     if ~strcmp(f32IntegGain_bkup,'0')
      |       set_param(gcb,'f32IntegGain','0');
      |     end
      |   else
      |     tmps=num2str(f32IntegGain);
      |     if ~strcmp(f32IntegGain_bkup,tmps)
      |       set_param(gcb,'f32IntegGain',tmps);
      |     end
      |   end
      |   if isnan(s16PropGainShift)
      |     if ~strcmp(s16PropGainShift_bkup,'0')
      |       set_param(gcb,'s16PropGainShift','0');
      |     end
      |   else
      |     tmps=num2str(s16PropGainShift);
      |     if ~strcmp(s16PropGainShift_bkup,tmps)
      |       set_param(gcb,'s16PropGainShift',tmps);
      |     end
      |   end
      |   if isnan(s16IntegGainShift)
      |     if ~strcmp(s16IntegGainShift_bkup,'0')
      |       set_param(gcb,'s16IntegGainShift','0');
      |     end
      |   else
      |     tmps=num2str(s16IntegGainShift);
      |     if ~strcmp(s16IntegGainShift_bkup,tmps)
      |       set_param(gcb,'s16IntegGainShift',tmps);
      |     end
      |   end
      |   if isnan(f32LowerLimit)
      |     if ~strcmp(f32LowerLimit_bkup,'0')
      |       set_param(gcb,'f32LowerLimit','0');
      |     end
      |   else
      |     tmps=num2str(f32LowerLimit);
      |     if ~strcmp(f32LowerLimit_bkup,tmps)
      |       set_param(gcb,'f32LowerLimit',tmps);
      |     end
      |   end
      |   if isnan(f32UpperLimit)
      |     if ~strcmp(f32UpperLimit_bkup,'0')
      |       set_param(gcb,'f32UpperLimit','0');
      |     end
      |   else
      |     tmps=num2str(f32UpperLimit);
      |     if ~strcmp(f32UpperLimit_bkup,tmps)
      |       set_param(gcb,'f32UpperLimit',tmps);
      |     end
      |   end
      | end
      mask Callback Idmax:
      | autoCalcEn=get_param(gcb,'autoCalcEn');
      | if strcmp(autoCalcEn,'on')
      |   SampleTime=Simulink.data.evalinGlobal(bdroot,get_param(gcb,'SampleTime'));
      |   if (SampleTime==-1)
      |     SampleTime=str2double(get_param(gcb,'SampleTime_1'));
      |   end
      |   u16NSamples_bkup=get_param(gcb,'u16NSamples');
      |   f32PropGain_bkup=get_param(gcb,'f32PropGain');
      |   f32IntegGain_bkup=get_param(gcb,'f32IntegGain');
      |   s16PropGainShift_bkup=get_param(gcb,'s16PropGainShift');
      |   s16IntegGainShift_bkup=get_param(gcb,'s16IntegGainShift');
      |   f32LowerLimit_bkup=get_param(gcb,'f32LowerLimit');
      |   f32UpperLimit_bkup=get_param(gcb,'f32UpperLimit');
      |   wf0=Simulink.data.evalinGlobal(bdroot,get_param(gcb,'wf0'));
      |   wksi=Simulink.data.evalinGlobal(bdroot,get_param(gcb,'wksi'));
      |   J=Simulink.data.evalinGlobal(bdroot,get_param(gcb,'J'));
      |   Kt=Simulink.data.evalinGlobal(bdroot,get_param(gcb,'Kt'));
      |   lambdaFW=Simulink.data.evalinGlobal(bdroot,get_param(gcb,'lambdaFW'));
      |   Idmax=Simulink.data.evalinGlobal(bdroot,get_param(gcb,'Idmax'));
      |   mechspeed=Simulink.data.evalinGlobal(bdroot,get_param(gcb,'mechspeed'));
      |   polepairs=Simulink.data.evalinGlobal(bdroot,get_param(gcb,'polepairs'));
      |   uscale=Simulink.data.evalinGlobal(bdroot,get_param(gcb,'uscale'));
      |   iscale=Simulink.data.evalinGlobal(bdroot,get_param(gcb,'iscale'));
      |   if (wf0<=0)
      |     warning('Natural frequency f0 must be positive.');
      |   end
      |   if (wksi<=0)
      |     warning('Current loop attenuation must be positive.');
      |   end
      |   if (wksi>1)
      |     warning('Current loop attenuation must not exceed 1.');
      |   end
      |   if (J<=0)
      |     warning('Moment of inertia J must be positive.');
      |   end
      |   if (Kt<=0)
      |     warning('Torque constant Kt must be positive.');
      |   end
      |   if (lambdaFW<0)
      |     warning('MA filter smoothing factor must be in the range 0..1.');
      |   end
      |   if (lambdaFW>1)
      |     warning('MA filter smoothing factor must be in the range 0..1.');
      |   end
      |   if (mechspeed<=0)
      |     warning('Max. speed must be positive.');
      |   end
      |   if (polepairs<1)
      |     warning('Number of pole pairs must be a natural number (1, 2, 3, ...).');
      |   end
      |   if (round(polepairs)~=polepairs)
      |     warning('Number of pole pairs must be a natural number (1, 2, 3, ...).');
      |   end
      |   if (uscale<=0)
      |     warning('U_max must be positive.');
      |   end
      |   if (iscale<=0)
      |     warning('I_max must be positive.');
      |   end
      |   w0=6.283185307179586*wf0;
      |   pgain=2.0*wksi*w0*J/Kt;
      |   igain=w0*w0*J/Kt;
      |   wmax=polepairs*mechspeed*0.1047197551196598;
      |   kif=igain*SampleTime*0.5*wmax/iscale;
      |   fwkpf=0.9*pgain*wmax/iscale;
      |   s16PropGainShift=ceil(log2(abs(fwkpf)));
      |   if s16PropGainShift<-31
      |     s16PropGainShift=-31;
      |   end
      |   if s16PropGainShift>31
      |     s16PropGainShift=31;
      |     warning(['Parameter s16PropGainShift of ' gcb ' exceeds the fixed-point range.']);
      |   end
      |   f32PropGain=round(fwkpf*2^(-s16PropGainShift)*2^31);
      |   if f32PropGain>2^31-1
      |     f32PropGain=2^31-1;
      |     warning(['Parameter f32PropGain of ' gcb ' exceeds the fixed-point range.']);
      |   end
      |   if f32PropGain<-2^31
      |     f32PropGain=-2^31;
      |     warning(['Parameter f32PropGain of ' gcb ' exceeds the fixed-point range.']);
      |   end
      |   s16IntegGainShift=ceil(log2(abs(kif)));
      |   if s16IntegGainShift<-31
      |     s16IntegGainShift=-31;
      |   end
      |   if s16IntegGainShift>31
      |     s16IntegGainShift=31;
      |     warning(['Parameter s16IntegGainShift of ' gcb ' exceeds the fixed-point range.']);
      |   end
      |   f32IntegGain=round(kif*2^(-s16IntegGainShift)*2^31);
      |   if f32IntegGain>2^31-1
      |     f32IntegGain=2^31-1;
      |     warning(['Parameter f32IntegGain of ' gcb ' exceeds the fixed-point range.']);
      |   end
      |   if f32IntegGain<-2^31
      |     f32IntegGain=-2^31;
      |     warning(['Parameter f32IntegGain of ' gcb ' exceeds the fixed-point range.']);
      |   end
      |   if (Idmax<0)
      |     iratio=abs(Idmax)/iscale;
      |     lowlim=0.3183098861837907*acos(iratio)-0.5;
      |   else
      |     lowlim=0.0;
      |   end
      |   f32LowerLimit=round(lowlim*2^31);
      |   if f32LowerLimit>2^31-1
      |     f32LowerLimit=2^31-1;
      |     warning(['Parameter f32LowerLimit of ' gcb ' exceeds the fixed-point range.']);
      |   end
      |   if f32LowerLimit<-2^31
      |     f32LowerLimit=-2^31;
      |     warning(['Parameter f32LowerLimit of ' gcb ' exceeds the fixed-point range.']);
      |   end
      |   f32UpperLimit=0;
      |   u16NSamples=round(log2(1.0/abs(lambdaFW)));
      |   if u16NSamples>31
      |     u16NSamples=31;
      |   end
      |   if u16NSamples<0
      |     u16NSamples=0;
      |   end
      |   if isnan(u16NSamples)
      |     if ~strcmp(u16NSamples_bkup,'0')
      |       set_param(gcb,'u16NSamples','0');
      |     end
      |   else
      |     tmps=num2str(u16NSamples);
      |     if ~strcmp(u16NSamples_bkup,tmps)
      |       set_param(gcb,'u16NSamples',tmps);
      |     end
      |   end
      |   if isnan(f32PropGain)
      |     if ~strcmp(f32PropGain_bkup,'0')
      |       set_param(gcb,'f32PropGain','0');
      |     end
      |   else
      |     tmps=num2str(f32PropGain);
      |     if ~strcmp(f32PropGain_bkup,tmps)
      |       set_param(gcb,'f32PropGain',tmps);
      |     end
      |   end
      |   if isnan(f32IntegGain)
      |     if ~strcmp(f32IntegGain_bkup,'0')
      |       set_param(gcb,'f32IntegGain','0');
      |     end
      |   else
      |     tmps=num2str(f32IntegGain);
      |     if ~strcmp(f32IntegGain_bkup,tmps)
      |       set_param(gcb,'f32IntegGain',tmps);
      |     end
      |   end
      |   if isnan(s16PropGainShift)
      |     if ~strcmp(s16PropGainShift_bkup,'0')
      |       set_param(gcb,'s16PropGainShift','0');
      |     end
      |   else
      |     tmps=num2str(s16PropGainShift);
      |     if ~strcmp(s16PropGainShift_bkup,tmps)
      |       set_param(gcb,'s16PropGainShift',tmps);
      |     end
      |   end
      |   if isnan(s16IntegGainShift)
      |     if ~strcmp(s16IntegGainShift_bkup,'0')
      |       set_param(gcb,'s16IntegGainShift','0');
      |     end
      |   else
      |     tmps=num2str(s16IntegGainShift);
      |     if ~strcmp(s16IntegGainShift_bkup,tmps)
      |       set_param(gcb,'s16IntegGainShift',tmps);
      |     end
      |   end
      |   if isnan(f32LowerLimit)
      |     if ~strcmp(f32LowerLimit_bkup,'0')
      |       set_param(gcb,'f32LowerLimit','0');
      |     end
      |   else
      |     tmps=num2str(f32LowerLimit);
      |     if ~strcmp(f32LowerLimit_bkup,tmps)
      |       set_param(gcb,'f32LowerLimit',tmps);
      |     end
      |   end
      |   if isnan(f32UpperLimit)
      |     if ~strcmp(f32UpperLimit_bkup,'0')
      |       set_param(gcb,'f32UpperLimit','0');
      |     end
      |   else
      |     tmps=num2str(f32UpperLimit);
      |     if ~strcmp(f32UpperLimit_bkup,tmps)
      |       set_param(gcb,'f32UpperLimit',tmps);
      |     end
      |   end
      | end
      mask Callback mechspeed:
      | autoCalcEn=get_param(gcb,'autoCalcEn');
      | if strcmp(autoCalcEn,'on')
      |   SampleTime=Simulink.data.evalinGlobal(bdroot,get_param(gcb,'SampleTime'));
      |   if (SampleTime==-1)
      |     SampleTime=str2double(get_param(gcb,'SampleTime_1'));
      |   end
      |   u16NSamples_bkup=get_param(gcb,'u16NSamples');
      |   f32PropGain_bkup=get_param(gcb,'f32PropGain');
      |   f32IntegGain_bkup=get_param(gcb,'f32IntegGain');
      |   s16PropGainShift_bkup=get_param(gcb,'s16PropGainShift');
      |   s16IntegGainShift_bkup=get_param(gcb,'s16IntegGainShift');
      |   f32LowerLimit_bkup=get_param(gcb,'f32LowerLimit');
      |   f32UpperLimit_bkup=get_param(gcb,'f32UpperLimit');
      |   wf0=Simulink.data.evalinGlobal(bdroot,get_param(gcb,'wf0'));
      |   wksi=Simulink.data.evalinGlobal(bdroot,get_param(gcb,'wksi'));
      |   J=Simulink.data.evalinGlobal(bdroot,get_param(gcb,'J'));
      |   Kt=Simulink.data.evalinGlobal(bdroot,get_param(gcb,'Kt'));
      |   lambdaFW=Simulink.data.evalinGlobal(bdroot,get_param(gcb,'lambdaFW'));
      |   Idmax=Simulink.data.evalinGlobal(bdroot,get_param(gcb,'Idmax'));
      |   mechspeed=Simulink.data.evalinGlobal(bdroot,get_param(gcb,'mechspeed'));
      |   polepairs=Simulink.data.evalinGlobal(bdroot,get_param(gcb,'polepairs'));
      |   uscale=Simulink.data.evalinGlobal(bdroot,get_param(gcb,'uscale'));
      |   iscale=Simulink.data.evalinGlobal(bdroot,get_param(gcb,'iscale'));
      |   if (wf0<=0)
      |     warning('Natural frequency f0 must be positive.');
      |   end
      |   if (wksi<=0)
      |     warning('Current loop attenuation must be positive.');
      |   end
      |   if (wksi>1)
      |     warning('Current loop attenuation must not exceed 1.');
      |   end
      |   if (J<=0)
      |     warning('Moment of inertia J must be positive.');
      |   end
      |   if (Kt<=0)
      |     warning('Torque constant Kt must be positive.');
      |   end
      |   if (lambdaFW<0)
      |     warning('MA filter smoothing factor must be in the range 0..1.');
      |   end
      |   if (lambdaFW>1)
      |     warning('MA filter smoothing factor must be in the range 0..1.');
      |   end
      |   if (mechspeed<=0)
      |     warning('Max. speed must be positive.');
      |   end
      |   if (polepairs<1)
      |     warning('Number of pole pairs must be a natural number (1, 2, 3, ...).');
      |   end
      |   if (round(polepairs)~=polepairs)
      |     warning('Number of pole pairs must be a natural number (1, 2, 3, ...).');
      |   end
      |   if (uscale<=0)
      |     warning('U_max must be positive.');
      |   end
      |   if (iscale<=0)
      |     warning('I_max must be positive.');
      |   end
      |   w0=6.283185307179586*wf0;
      |   pgain=2.0*wksi*w0*J/Kt;
      |   igain=w0*w0*J/Kt;
      |   wmax=polepairs*mechspeed*0.1047197551196598;
      |   kif=igain*SampleTime*0.5*wmax/iscale;
      |   fwkpf=0.9*pgain*wmax/iscale;
